simulink library "ammclib_bam_S32K14x"  (R2016a)
settings: Solver=VariableStepAuto  SolverMode=SingleTasking  StartTime=0.0  StopTime=10.0  RelTol=1e-3
undefined symbols (not defined in the file or in its folder): f16A1, f16A2, f16ADCMaxError, f16B0, f16B1, f16B2, f16C1, f16CC1, f16CC1sc, f16CC1sc_D, f16CC1sc_Q, f16CC2, f16CC2sc, f16CC2sc_D, f16CC2sc_Q, f16DerivGain, f16EGain, f16FiltCoef, f16HystOff, f16HystOn, f16IGain, f16IntegGain, f16IntegGainFW, f16IntegGainQ, f16Kd, f16Kq, f16Limit, f16LowerLimit, f16LowerLimit_D, f16LowerLimit_Q, f16LowerLimitFW, f16LowerLimitQ, f16ModIndex, f16OutValOff, f16OutValOn, f16PropGain, f16PropGainFW, f16PropGainQ, f16RampDown, f16RampUp, f16UGain, f16UpperLimit, f16UpperLimit_D, f16UpperLimit_Q, f16UpperLimitFW, f16UpperLimitQ, f16WIGain, f32A1, f32A2, f32ADCMaxError, f32B0, f32B1, f32B2, f32C1, f32CC1, f32CC1sc, f32CC1sc_D, f32CC1sc_Q, f32CC2, f32CC2sc ... (+114)
(part 6 of 22)

== system ammclib_bam_S32K14x/AMCLIB/FLT ==
  AMCLIB_BemfObsrvDQ_FLT : Subsystem  TreatAsAtomicUnit=on  mask(AMCLIB_BemfObsrvDQ_FLT){showStates=Hide (faster execution), resetStatesEnable=Pre-set according to the first set of inputs after reset, fltIGain=0, fltUGain=0, fltWIGain=0, fltEGain=0, fltCC1sc_D=0, fltCC2sc_D=0, fltUpperLimit_D=0, fltLowerLimit_D=0, fltCC1sc_Q=0, fltCC2sc_Q=0, fltUpperLimit_Q=0, fltLowerLimit_Q=0}
      mask prompts: showStates "Show internal states"; resetStatesEnable "Internal state after reset"; fltIGain "fltIGain (RL circuit constant)"; fltUGain "fltUGain (Voltage cross-coupling constant)"; fltWIGain "fltWIGain (Angular velocity cross-coupling constant)"; fltEGain "fltEGain (Back-EMF cross-coupling constant)"; fltCC1sc_D "fltCC1sc_D (CC1 coefficient of the D-axis PI controller)"; fltCC2sc_D "fltCC2sc_D (CC2 coefficient of the D-axis PI controller)"; fltUpperLimit_D "fltUpperLimit_D (Upper Limit of the D-axis PI controller)"; fltLowerLimit_D "fltLowerLimit_D (Lower Limit of the D-axis PI controller)"; fltCC1sc_Q "fltCC1sc_Q (CC1 coefficient of the Q-axis PI controller)"; fltCC2sc_Q "fltCC2sc_Q (CC2 coefficient of the Q-axis PI controller)"; fltUpperLimit_Q "fltUpperLimit_Q (Upper Limit of the Q-axis PI controller)"; fltLowerLimit_Q "fltLowerLimit_Q (Lower Limit of the Q-axis PI controller)"
      mask help: PMSM back-EMF observer DQ in single precision floating-point implementation. This block supports re-initialization of the internal state during simulation. If the block is reset, the observer will align with the motor's position and speed measured in the next time step. This allows seamless on-the-fly transition to the closed-loop control. Refer to the AMMCLIB User's Guide for further details.
      mask init:
      | if ~evalin('base','exist(''tS8'',''var'')')
      |   if (2 ~= exist('SWLIBS_Typedefs.mat','file'))
      |       error('File SWLIBS_Typedefs.mat is not on the Matlab path. Please add the AMMCLIB "bam" folder in the Matlab Search Path.');
      |   else
      |       evalin('base', 'load(''SWLIBS_Typedefs.mat'')');
      |   end
      | end
      | if showStates == 1
      |     % hidden state variables
      |     if strcmp(get_param([gcb '/fltIGain'], 'BlockType'), 'Inport')
      |         posblk = get_param(gcb, 'Position');
      | 
      |         pos = get_param(    [gcb, '/fltIGain'], 'Position');
      |         orient = get_param( [gcb, '/fltIGain'], 'Orientation');
      |         delete_block(       [gcb, '/fltIGain']);
      |         add_block('built-in/Ground', [gcb, '/fltIGain'], 'Position', pos, 'Orientation', orient);
      | 
      |         pos = get_param(    [gcb, '/fltUGain'], 'Position');
      |         orient = get_param( [gcb, '/fltUGain'], 'Orientation');
      |         delete_block(       [gcb, '/fltUGain']);
      |         add_block('built-in/Ground', [gcb, '/fltUGain'], 'Position', pos, 'Orientation', orient);
      | 
      |         pos = get_param(    [gcb, '/fltWIGain'], 'Position');
      |         orient = get_param( [gcb, '/fltWIGain'], 'Orientation');
      |         delete_block(       [gcb, '/fltWIGain']);
      |         add_block('built-in/Ground', [gcb, '/fltWIGain'], 'Position', pos, 'Orientation', orient);
      | 
      |         pos = get_param(    [gcb, '/fltEGain'], 'Position');
      |         orient = get_param( [gcb, '/fltEGain'], 'Orientation');
      |         delete_block(       [gcb, '/fltEGain']);
      |         add_block('built-in/Ground', [gcb, '/fltEGain'], 'Position', pos, 'Orientation', orient);
      | 
      |         pos = get_param(    [gcb, '/fltCC1sc_D'], 'Position');
      |         orient = get_param( [gcb, '/fltCC1sc_D'], 'Orientation');
      |         delete_block(       [gcb, '/fltCC1sc_D']);
      |         add_block('built-in/Ground', [gcb, '/fltCC1sc_D'], 'Position', pos, 'Orientation', orient);
      | 
      |         pos = get_param(    [gcb, '/fltCC2sc_D'], 'Position');
      |         orient = get_param( [gcb, '/fltCC2sc_D'], 'Orientation');
      |         delete_block(       [gcb, '/fltCC2sc_D']);
      |         add_block('built-in/Ground', [gcb, '/fltCC2sc_D'], 'Position', pos, 'Orientation', orient);
      | 
      |         pos = get_param(    [gcb, '/fltUpperLimit_D'], 'Position');
      |         orient = get_param( [gcb, '/fltUpperLimit_D'], 'Orientation');
      |         delete_block(       [gcb, '/fltUpperLimit_D']);
      |         add_block('built-in/Ground', [gcb, '/fltUpperLimit_D'], 'Position', pos, 'Orientation', orient);
      | 
      |         pos = get_param(    [gcb, '/fltLowerLimit_D'], 'Position');
      |         orient = get_param( [gcb, '/fltLowerLimit_D'], 'Orientation');
      |         delete_block(       [gcb, '/fltLowerLimit_D']);
      |         add_block('built-in/Ground', [gcb, '/fltLowerLimit_D'], 'Position', pos, 'Orientation', orient);
      | 
      |         pos = get_param(    [gcb, '/fltCC1sc_Q'], 'Position');
      |         orient = get_param( [gcb, '/fltCC1sc_Q'], 'Orientation');
      |         delete_block(       [gcb, '/fltCC1sc_Q']);
      |         add_block('built-in/Ground', [gcb, '/fltCC1sc_Q'], 'Position', pos, 'Orientation', orient);
      | 
      |         pos = get_param(    [gcb, '/fltCC2sc_Q'], 'Position');
      |         orient = get_param( [gcb, '/fltCC2sc_Q'], 'Orientation');
      |         delete_block(       [gcb, '/fltCC2sc_Q']);
      |         add_block('built-in/Ground', [gcb, '/fltCC2sc_Q'], 'Position', pos, 'Orientation', orient);
      | 
      |         pos = get_param(    [gcb, '/fltUpperLimit_Q'], 'Position');
      |         orient = get_param( [gcb, '/fltUpperLimit_Q'], 'Orientation');
      |         delete_block(       [gcb, '/fltUpperLimit_Q']);
      |         add_block('built-in/Ground', [gcb, '/fltUpperLimit_Q'], 'Position', pos, 'Orientation', orient);
      | 
      |         pos = get_param(    [gcb, '/fltLowerLimit_Q'], 'Position');
      |         orient = get_param( [gcb, '/fltLowerLimit_Q'], 'Orientation');
      |         delete_block(       [gcb, '/fltLowerLimit_Q']);
      |         add_block('built-in/Ground', [gcb, '/fltLowerLimit_Q'], 'Position', pos, 'Orientation', orient);
      | 
      |         pos = get_param(    [gcb, '/fltAcc_D'], 'Position');
      |         orient = get_param( [gcb, '/fltAcc_D'], 'Orientation');
      |         delete_block(       [gcb, '/fltAcc_D']);
      |         add_block('built-in/Ground', [gcb, '/fltAcc_D'], 'Position', pos, 'Orientation', orient);
      | 
      |         pos = get_param(    [gcb, '/fltInErrK1_D'], 'Position');
      |         orient = get_param( [gcb, '/fltInErrK1_D'], 'Orientation');
      |         delete_block(       [gcb, '/fltInErrK1_D']);
      |         add_block('built-in/Ground', [gcb, '/fltInErrK1_D'], 'Position', pos, 'Orientation', orient);
      | 
      |         pos = get_param(    [gcb, '/fltAcc_Q'], 'Position');
      |         orient = get_param( [gcb, '/fltAcc_Q'], 'Orientation');
      |         delete_block(       [gcb, '/fltAcc_Q']);
      |         add_block('built-in/Ground', [gcb, '/fltAcc_Q'], 'Position', pos, 'Orientation', orient);
      | 
      |         pos = get_param(    [gcb, '/fltInErrK1_Q'], 'Position');
      |         orient = get_param( [gcb, '/fltInErrK1_Q'], 'Orientation');
      |         delete_block(       [gcb, '/fltInErrK1_Q']);
      |         add_block('built-in/Ground', [gcb, '/fltInErrK1_Q'], 'Position', pos, 'Orientation', orient);
      | 
      |         pos = get_param(    [gcb, '/fltIObsrvIn_1_D'], 'Position');
      |         orient = get_param( [gcb, '/fltIObsrvIn_1_D'], 'Orientation');
      |         delete_block(       [gcb, '/fltIObsrvIn_1_D']);
      |         add_block('built-in/Ground', [gcb, '/fltIObsrvIn_1_D'], 'Position', pos, 'Orientation', orient);
      | 
      |         pos = get_param(    [gcb, '/fltIObsrvIn_1_Q'], 'Position');
      |         orient = get_param( [gcb, '/fltIObsrvIn_1_Q'], 'Orientation');
      |         delete_block(       [gcb, '/fltIObsrvIn_1_Q']);
      |         add_block('built-in/Ground', [gcb, '/fltIObsrvIn_1_Q'], 'Position', pos, 'Orientation', orient);
      | 
      |         pos = get_param(    [gcb, '/fltIObsrv_D'], 'Position');
      |         orient = get_param( [gcb, '/fltIObsrv_D'], 'Orientation');
      |         delete_block(       [gcb, '/fltIObsrv_D']);
      |         add_block('built-in/Ground', [gcb, '/fltIObsrv_D'], 'Position', pos, 'Orientation', orient);
      | 
      |         pos = get_param(    [gcb, '/fltIObsrv_Q'], 'Position');
      |         orient = get_param( [gcb, '/fltIObsrv_Q'], 'Orientation');
      |         delete_block(       [gcb, '/fltIObsrv_Q']);
      |         add_block('built-in/Ground', [gcb, '/fltIObsrv_Q'], 'Position', pos, 'Orientation', orient);
      | 
      | 
      |         pos = get_param(    [gcb '/fltEObsrv_D_Out'], 'Position');
      |         orient = get_param( [gcb '/fltEObsrv_D_Out'], 'Orientation');
      |         delete_block(       [gcb '/fltEObsrv_D_Out']);
      |         add_block('built-in/Terminator', [gcb '/fltEObsrv_D_Out'], 'Position', pos, 'Orientation', orient);
      | 
      |         pos = get_param(    [gcb '/fltEObsrv_Q_Out'], 'Position');
      |         orient = get_param( [gcb '/fltEObsrv_Q_Out'], 'Orientation');
      |         delete_block(       [gcb '/fltEObsrv_Q_Out']);
      |         add_block('built-in/Terminator', [gcb '/fltEObsrv_Q_Out'], 'Position', pos, 'Orientation', orient);
      | 
      |         pos = get_param(    [gcb '/fltAcc_D_Out'], 'Position');
      |         orient = get_param( [gcb '/fltAcc_D_Out'], 'Orientation');
      |         delete_block(       [gcb '/fltAcc_D_Out']);
      |         add_block('built-in/Terminator', [gcb '/fltAcc_D_Out'], 'Position', pos, 'Orientation', orient);
      | 
      |         pos = get_param(    [gcb '/fltInErrK1_D_Out'], 'Position');
      |         orient = get_param( [gcb '/fltInErrK1_D_Out'], 'Orientation');
      |         delete_block(       [gcb '/fltInErrK1_D_Out']);
      |         add_block('built-in/Terminator', [gcb '/fltInErrK1_D_Out'], 'Position', pos, 'Orientation', orient);
      | 
      |         pos = get_param(    [gcb '/fltAcc_Q_Out'], 'Position');
      |         orient = get_param( [gcb '/fltAcc_Q_Out'], 'Orientation');
      |         delete_block(       [gcb '/fltAcc_Q_Out']);
      |         add_block('built-in/Terminator', [gcb '/fltAcc_Q_Out'], 'Position', pos, 'Orientation', orient);
      | 
      |         pos = get_param(    [gcb '/fltInErrK1_Q_Out'], 'Position');
      |         orient = get_param( [gcb '/fltInErrK1_Q_Out'], 'Orientation');
      |         delete_block(       [gcb '/fltInErrK1_Q_Out']);
      |         add_block('built-in/Terminator', [gcb '/fltInErrK1_Q_Out'], 'Position', pos, 'Orientation', orient);
      | 
      |         pos = get_param(    [gcb '/fltIObsrvIn_1_D_Out'], 'Position');
      |         orient = get_param( [gcb '/fltIObsrvIn_1_D_Out'], 'Orientation');
      |         delete_block(       [gcb '/fltIObsrvIn_1_D_Out']);
      |         add_block('built-in/Terminator', [gcb '/fltIObsrvIn_1_D_Out'], 'Position', pos, 'Orientation', orient);
      | 
      |         pos = get_param(    [gcb '/fltIObsrvIn_1_Q_Out'], 'Position');
      |         orient = get_param( [gcb '/fltIObsrvIn_1_Q_Out'], 'Orientation');
      |         delete_block(       [gcb '/fltIObsrvIn_1_Q_Out']);
      |         add_block('built-in/Terminator', [gcb '/fltIObsrvIn_1_Q_Out'], 'Position', pos, 'Orientation', orient);
      | 
      |         pos = get_param(    [gcb '/fltIObsrv_D_Out'], 'Position');
      |         orient = get_param( [gcb '/fltIObsrv_D_Out'], 'Orientation');
      |         delete_block(       [gcb '/fltIObsrv_D_Out']);
      |         add_block('built-in/Terminator', [gcb '/fltIObsrv_D_Out'], 'Position', pos, 'Orientation', orient);
      | 
      |         pos = get_param(    [gcb '/fltIObsrv_Q_Out'], 'Position');
      |         orient = get_param( [gcb '/fltIObsrv_Q_Out'], 'Orientation');
      |         delete_block(       [gcb '/fltIObsrv_Q_Out']);
      |         add_block('built-in/Terminator', [gcb '/fltIObsrv_Q_Out'], 'Position', pos, 'Orientation', orient);
      | 
      | 
      |         set_param([gcb '/pIAB'], 'Port', '1');
      |         set_param([gcb '/pUAB'], 'Port', '2');
      |         set_param([gcb '/fltVelocity'], 'Port', '3');
      |         set_param([gcb '/fltPhase'], 'Port', '4');
      | 
      |         set_param([gcb '/fltPhaseErr'], 'Port', '1');
      | 
      |         set_param(gcb,'MaskEnables',{'on','on','on','on','on','on','on','on','on','on','on','on','on','on'});
      | 
      |         if (posblk(4) - posblk(2)) > 125
      |           height = 125;
      |           set_param(gcb,'Position',[posblk(1), posblk(2), posblk(3), posblk(2)+height])
      |         end
      |     end
      | else
      |     % shown state variables
      |     if strcmp(get_param([gcb '/fltIGain'], 'BlockType'), 'Ground')
      |         posblk = get_param(gcb, 'Position');
      | 
      |         pos = get_param(    [gcb, '/fltIGain'], 'Position');
      |         orient = get_param( [gcb, '/fltIGain'], 'Orientation');
      |         delete_block(       [gcb, '/fltIGain']);
      |         add_block('built-in/Inport', [gcb, '/fltIGain'], 'Position', pos, 'Orientation', orient, 'OutDataTypeStr', 'single');
      | 
      |         pos = get_param(    [gcb, '/fltUGain'], 'Position');
      |         orient = get_param( [gcb, '/fltUGain'], 'Orientation');
      |         delete_block(       [gcb, '/fltUGain']);
      |         add_block('built-in/Inport', [gcb, '/fltUGain'], 'Position', pos, 'Orientation', orient, 'OutDataTypeStr', 'single');
      | 
      |         pos = get_param(    [gcb, '/fltWIGain'], 'Position');
      |         orient = get_param( [gcb, '/fltWIGain'], 'Orientation');
      |         delete_block(       [gcb, '/fltWIGain']);
      |         add_block('built-in/Inport', [gcb, '/fltWIGain'], 'Position', pos, 'Orientation', orient, 'OutDataTypeStr', 'single');
      | 
      |         pos = get_param(    [gcb, '/fltEGain'], 'Position');
      |         orient = get_param( [gcb, '/fltEGain'], 'Orientation');
      |         delete_block(       [gcb, '/fltEGain']);
      |         add_block('built-in/Inport', [gcb, '/fltEGain'], 'Position', pos, 'Orientation', orient, 'OutDataTypeStr', 'single');
      | 
      |         pos = get_param(    [gcb, '/fltCC1sc_D'], 'Position');
      |         orient = get_param( [gcb, '/fltCC1sc_D'], 'Orientation');
      |         delete_block(       [gcb, '/fltCC1sc_D']);
      |         add_block('built-in/Inport', [gcb, '/fltCC1sc_D'], 'Position', pos, 'Orientation', orient, 'OutDataTypeStr', 'single');
      | 
      |         pos = get_param(    [gcb, '/fltCC2sc_D'], 'Position');
      |         orient = get_param( [gcb, '/fltCC2sc_D'], 'Orientation');
      |         delete_block(       [gcb, '/fltCC2sc_D']);
      |         add_block('built-in/Inport', [gcb, '/fltCC2sc_D'], 'Position', pos, 'Orientation', orient, 'OutDataTypeStr', 'single');
      | 
      |         pos = get_param(    [gcb, '/fltUpperLimit_D'], 'Position');
      |         orient = get_param( [gcb, '/fltUpperLimit_D'], 'Orientation');
      |         delete_block(       [gcb, '/fltUpperLimit_D']);
      |         add_block('built-in/Inport', [gcb, '/fltUpperLimit_D'], 'Position', pos, 'Orientation', orient, 'OutDataTypeStr', 'single');
      | 
      |         pos = get_param(    [gcb, '/fltLowerLimit_D'], 'Position');
      |         orient = get_param( [gcb, '/fltLowerLimit_D'], 'Orientation');
      |         delete_block(       [gcb, '/fltLowerLimit_D']);
      |         add_block('built-in/Inport', [gcb, '/fltLowerLimit_D'], 'Position', pos, 'Orientation', orient, 'OutDataTypeStr', 'single');
      | 
      |         pos = get_param(    [gcb, '/fltCC1sc_Q'], 'Position');
      |         orient = get_param( [gcb, '/fltCC1sc_Q'], 'Orientation');
      |         delete_block(       [gcb, '/fltCC1sc_Q']);
      |         add_block('built-in/Inport', [gcb, '/fltCC1sc_Q'], 'Position', pos, 'Orientation', orient, 'OutDataTypeStr', 'single');
      | 
      |         pos = get_param(    [gcb, '/fltCC2sc_Q'], 'Position');
      |         orient = get_param( [gcb, '/fltCC2sc_Q'], 'Orientation');
      |         delete_block(       [gcb, '/fltCC2sc_Q']);
      |         add_block('built-in/Inport', [gcb, '/fltCC2sc_Q'], 'Position', pos, 'Orientation', orient, 'OutDataTypeStr', 'single');
      | 
      |         pos = get_param(    [gcb, '/fltUpperLimit_Q'], 'Position');
      |         orient = get_param( [gcb, '/fltUpperLimit_Q'], 'Orientation');
      |         delete_block(       [gcb, '/fltUpperLimit_Q']);
      |         add_block('built-in/Inport', [gcb, '/fltUpperLimit_Q'], 'Position', pos, 'Orientation', orient, 'OutDataTypeStr', 'single');
      | 
      |         pos = get_param(    [gcb, '/fltLowerLimit_Q'], 'Position');
      |         orient = get_param( [gcb, '/fltLowerLimit_Q'], 'Orientation');
      |         delete_block(       [gcb, '/fltLowerLimit_Q']);
      |         add_block('built-in/Inport', [gcb, '/fltLowerLimit_Q'], 'Position', pos, 'Orientation', orient, 'OutDataTypeStr', 'single');
      | 
      |         pos = get_param(    [gcb, '/fltAcc_D'], 'Position');
      |         orient = get_param( [gcb, '/fltAcc_D'], 'Orientation');
      |         delete_block(       [gcb, '/fltAcc_D']);
      |         add_block('built-in/Inport', [gcb, '/fltAcc_D'], 'Position', pos, 'Orientation', orient, 'OutDataTypeStr', 'single');
      | 
      |         pos = get_param(    [gcb, '/fltInErrK1_D'], 'Position');
      |         orient = get_param( [gcb, '/fltInErrK1_D'], 'Orientation');
      |         delete_block(       [gcb, '/fltInErrK1_D']);
      |         add_block('built-in/Inport', [gcb, '/fltInErrK1_D'], 'Position', pos, 'Orientation', orient, 'OutDataTypeStr', 'single');
      | 
      |         pos = get_param(    [gcb, '/fltAcc_Q'], 'Position');
      |         orient = get_param( [gcb, '/fltAcc_Q'], 'Orientation');
      |         delete_block(       [gcb, '/fltAcc_Q']);
      |         add_block('built-in/Inport', [gcb, '/fltAcc_Q'], 'Position', pos, 'Orientation', orient, 'OutDataTypeStr', 'single');
      | 
      |         pos = get_param(    [gcb, '/fltInErrK1_Q'], 'Position');
      |         orient = get_param( [gcb, '/fltInErrK1_Q'], 'Orientation');
      |         delete_block(       [gcb, '/fltInErrK1_Q']);
      |         add_block('built-in/Inport', [gcb, '/fltInErrK1_Q'], 'Position', pos, 'Orientation', orient, 'OutDataTypeStr', 'single');
      | 
      |         pos = get_param(    [gcb, '/fltIObsrvIn_1_D'], 'Position');
      |         orient = get_param( [gcb, '/fltIObsrvIn_1_D'], 'Orientation');
      |         delete_block(       [gcb, '/fltIObsrvIn_1_D']);
      |         add_block('built-in/Inport', [gcb, '/fltIObsrvIn_1_D'], 'Position', pos, 'Orientation', orient, 'OutDataTypeStr', 'single');
      | 
      |         pos = get_param(    [gcb, '/fltIObsrvIn_1_Q'], 'Position');
      |         orient = get_param( [gcb, '/fltIObsrvIn_1_Q'], 'Orientation');
      |         delete_block(       [gcb, '/fltIObsrvIn_1_Q']);
      |         add_block('built-in/Inport', [gcb, '/fltIObsrvIn_1_Q'], 'Position', pos, 'Orientation', orient, 'OutDataTypeStr', 'single');
      | 
      |         pos = get_param(    [gcb, '/fltIObsrv_D'], 'Position');
      |         orient = get_param( [gcb, '/fltIObsrv_D'], 'Orientation');
      |         delete_block(       [gcb, '/fltIObsrv_D']);
      |         add_block('built-in/Inport', [gcb, '/fltIObsrv_D'], 'Position', pos, 'Orientation', orient, 'OutDataTypeStr', 'single');
      | 
      |         pos = get_param(    [gcb, '/fltIObsrv_Q'], 'Position');
      |         orient = get_param( [gcb, '/fltIObsrv_Q'], 'Orientation');
      |         delete_block(       [gcb, '/fltIObsrv_Q']);
      |         add_block('built-in/Inport', [gcb, '/fltIObsrv_Q'], 'Position', pos, 'Orientation', orient, 'OutDataTypeStr', 'single');
      | 
      | 
      |         pos = get_param(    [gcb '/fltEObsrv_D_Out'], 'Position');
      |         orient = get_param( [gcb '/fltEObsrv_D_Out'], 'Orientation');
      |         delete_block(       [gcb '/fltEObsrv_D_Out']);
      |         add_block('built-in/Outport', [gcb '/fltEObsrv_D_Out'], 'Position', pos, 'Orientation', orient);
      | 
      |         pos = get_param(    [gcb '/fltEObsrv_Q_Out'], 'Position');
      |         orient = get_param( [gcb '/fltEObsrv_Q_Out'], 'Orientation');
      |         delete_block(       [gcb '/fltEObsrv_Q_Out']);
      |         add_block('built-in/Outport', [gcb '/fltEObsrv_Q_Out'], 'Position', pos, 'Orientation', orient);
      | 
      |         pos = get_param(    [gcb '/fltAcc_D_Out'], 'Position');
      |         orient = get_param( [gcb '/fltAcc_D_Out'], 'Orientation');
      |         delete_block(       [gcb '/fltAcc_D_Out']);
      |         add_block('built-in/Outport', [gcb '/fltAcc_D_Out'], 'Position', pos, 'Orientation', orient);
      | 
      |         pos = get_param(    [gcb '/fltInErrK1_D_Out'], 'Position');
      |         orient = get_param( [gcb '/fltInErrK1_D_Out'], 'Orientation');
      |         delete_block(       [gcb '/fltInErrK1_D_Out']);
      |         add_block('built-in/Outport', [gcb '/fltInErrK1_D_Out'], 'Position', pos, 'Orientation', orient);
      | 
      |         pos = get_param(    [gcb '/fltAcc_Q_Out'], 'Position');
      |         orient = get_param( [gcb '/fltAcc_Q_Out'], 'Orientation');
      |         delete_block(       [gcb '/fltAcc_Q_Out']);
      |         add_block('built-in/Outport', [gcb '/fltAcc_Q_Out'], 'Position', pos, 'Orientation', orient);
      | 
      |         pos = get_param(    [gcb '/fltInErrK1_Q_Out'], 'Position');
      |         orient = get_param( [gcb '/fltInErrK1_Q_Out'], 'Orientation');
      |         delete_block(       [gcb '/fltInErrK1_Q_Out']);
      |         add_block('built-in/Outport', [gcb '/fltInErrK1_Q_Out'], 'Position', pos, 'Orientation', orient);
      | 
      |         pos = get_param(    [gcb '/fltIObsrvIn_1_D_Out'], 'Position');
      |         orient = get_param( [gcb '/fltIObsrvIn_1_D_Out'], 'Orientation');
      |         delete_block(       [gcb '/fltIObsrvIn_1_D_Out']);
      |         add_block('built-in/Outport', [gcb '/fltIObsrvIn_1_D_Out'], 'Position', pos, 'Orientation', orient);
      | 
      |         pos = get_param(    [gcb '/fltIObsrvIn_1_Q_Out'], 'Position');
      |         orient = get_param( [gcb '/fltIObsrvIn_1_Q_Out'], 'Orientation');
      |         delete_block(       [gcb '/fltIObsrvIn_1_Q_Out']);
      |         add_block('built-in/Outport', [gcb '/fltIObsrvIn_1_Q_Out'], 'Position', pos, 'Orientation', orient);
      | 
      |         pos = get_param(    [gcb '/fltIObsrv_D_Out'], 'Position');
      |         orient = get_param( [gcb '/fltIObsrv_D_Out'], 'Orientation');
      |         delete_block(       [gcb '/fltIObsrv_D_Out']);
      |         add_block('built-in/Outport', [gcb '/fltIObsrv_D_Out'], 'Position', pos, 'Orientation', orient);
      | 
      |         pos = get_param(    [gcb '/fltIObsrv_Q_Out'], 'Position');
      |         orient = get_param( [gcb '/fltIObsrv_Q_Out'], 'Orientation');
      |         delete_block(       [gcb '/fltIObsrv_Q_Out']);
      |         add_block('built-in/Outport', [gcb '/fltIObsrv_Q_Out'], 'Position', pos, 'Orientation', orient);
      | 
      | 
      |         set_param([gcb '/pIAB'], 'Port', '1');
      |         set_param([gcb '/pUAB'], 'Port', '2');
      |         set_param([gcb '/fltVelocity'], 'Port', '3');
      |         set_param([gcb '/fltPhase'], 'Port', '4');
      |         set_param([gcb '/fltIGain'], 'Port', '5');
      |         set_param([gcb '/fltUGain'], 'Port', '6');
      |         set_param([gcb '/fltWIGain'], 'Port', '7');
      |         set_param([gcb '/fltEGain'], 'Port', '8');
      |         set_param([gcb '/fltCC1sc_D'], 'Port', '9');
      |         set_param([gcb '/fltCC2sc_D'], 'Port', '10');
      |         set_param([gcb '/fltUpperLimit_D'], 'Port', '11');
      |         set_param([gcb '/fltLowerLimit_D'], 'Port', '12');
      |         set_param([gcb '/fltCC1sc_Q'], 'Port', '13');
      |         set_param([gcb '/fltCC2sc_Q'], 'Port', '14');
      |         set_param([gcb '/fltUpperLimit_Q'], 'Port', '15');
      |         set_param([gcb '/fltLowerLimit_Q'], 'Port', '16');
      |         set_param([gcb '/fltAcc_D'], 'Port', '17');
      |         set_param([gcb '/fltInErrK1_D'], 'Port', '18');
      |         set_param([gcb '/fltAcc_Q'], 'Port', '19');
      |         set_param([gcb '/fltInErrK1_Q'], 'Port', '20');
      |         set_param([gcb '/fltIObsrvIn_1_D'], 'Port', '21');
      |         set_param([gcb '/fltIObsrvIn_1_Q'], 'Port', '22');
      |         set_param([gcb '/fltIObsrv_D'], 'Port', '23');
      |         set_param([gcb '/fltIObsrv_Q'], 'Port', '24');
      | 
      |         set_param([gcb '/fltPhaseErr'], 'Port', '1');
      |         set_param([gcb '/fltEObsrv_D_Out'], 'Port', '2');
      |         set_param([gcb '/fltEObsrv_Q_Out'], 'Port', '3');
      |         set_param([gcb '/fltAcc_D_Out'], 'Port', '4');
      |         set_param([gcb '/fltInErrK1_D_Out'], 'Port', '5');
      |         set_param([gcb '/fltAcc_Q_Out'], 'Port', '6');
      |         set_param([gcb '/fltInErrK1_Q_Out'], 'Port', '7');
      |         set_param([gcb '/fltIObsrvIn_1_D_Out'], 'Port', '8');
      |         set_param([gcb '/fltIObsrvIn_1_Q_Out'], 'Port', '9');
      |         set_param([gcb '/fltIObsrv_D_Out'], 'Port', '10');
      |         set_param([gcb '/fltIObsrv_Q_Out'], 'Port', '11');
      | 
      |         set_param(gcb,'MaskEnables',{'on','on','off','off','off','off','off','off','off','off','off','off','off','off'});
      | 
      |         if (posblk(4) - posblk(2)) < 625
      |           height = 625;
      |           set_param(gcb,'Position',[posblk(1), posblk(2), posblk(3), posblk(2)+height])
      |         end
      |     end
      | end
      settings: RTWSystemCode=Inline
      mask Help: web([fileparts(which('ammclib_bam_S32K14x.slx')) '/../doc/S32K14XMCLUG.pdf'], '-browser')
      mask TypeOptions showStates: Hide (faster execution) | Show (allows debugging; connect feedback loops manually)
      mask Callback showStates:
      | maskStr = get_param(gcb,'showStates');
      | if strcmp(maskStr,'Hide (faster execution)'),
      |     set_param(gcb,'MaskEnables',{'on','on','on','on','on','on','on','on','on','on','on','on','on','on'});
      | else
      |     set_param(gcb,'MaskEnables',{'on','on','off','off','off','off','off','off','off','off','off','off','off','off'});
      | end
      mask TypeOptions resetStatesEnable: Pre-set according to the first set of inputs after reset | Clear to zero
      mask Display:
      | color('black');
      | pos = get_param(gcb, 'Position');
      | width = pos(3) - pos(1);
      | height = pos(4) - pos(2);
      | tX=width/2;
      | tY=height - 25;
      | color('black');
      | text(tX,tY, 'AMCLIB_BemfObsrvDQ_FLT', 'horizontalAlignment', 'center');
      | if showStates == 2
      |   color('red');
      |   text(tX,tY - 20, ['debugging mode' char(13) char(10) '(limited performance)'], 'horizontalAlignment', 'center');
      | end
  AMCLIB_CurrentLoop_FLT : Subsystem  TreatAsAtomicUnit=on  mask(AMCLIB_CurrentLoop_FLT){showStates=Hide (faster execution), resetStatesEnable=Pre-set according to the first set of inputs after reset, fltCC1sc_D=0, fltCC2sc_D=0, fltCC1sc_Q=0, fltCC2sc_Q=0}
      mask prompts: showStates "Show internal states"; resetStatesEnable "Internal state after reset"; fltCC1sc_D "fltCC1sc_D (CC1 coefficient of the D-axis PI controller)"; fltCC2sc_D "fltCC2sc_D (CC2 coefficient of the D-axis PI controller)"; fltCC1sc_Q "fltCC1sc_Q (CC1 coefficient of the Q-axis PI controller)"; fltCC2sc_Q "fltCC2sc_Q (CC2 coefficient of the Q-axis PI controller)"
      mask help: Current control loop of the PMSM field-oriented control algorithm in single precision floating-point implementation. This block supports re-initialization of the internal state during simulation. If the block is reset, the outputs of the PI controllers will be aligned with the inputs fltControllerPIrAWDOut_preset and fltControllerPIrAWQOut_preset. Refer to the AMMCLIB User's Guide for further details.
      mask init:
      | if ~evalin('base','exist(''tS8'',''var'')')
      |   if (2 ~= exist('SWLIBS_Typedefs.mat','file'))
      |       error('File SWLIBS_Typedefs.mat is not on the Matlab path. Please add the AMMCLIB "bam" folder in the Matlab Search Path.');
      |   else
      |       evalin('base', 'load(''SWLIBS_Typedefs.mat'')');
      |   end
      | end
      | if showStates == 1
      |     % hidden state variables
      |     if strcmp(get_param([gcb '/fltCC1sc_D'], 'BlockType'), 'Inport')
      |         posblk = get_param(gcb, 'Position');
      | 
      |         pos = get_param(    [gcb, '/fltCC1sc_D'], 'Position');
      |         orient = get_param( [gcb, '/fltCC1sc_D'], 'Orientation');
      |         delete_block(       [gcb, '/fltCC1sc_D']);
      |         add_block('built-in/Ground', [gcb, '/fltCC1sc_D'], 'Position', pos, 'Orientation', orient);
      | 
      |         pos = get_param(    [gcb, '/fltCC2sc_D'], 'Position');
      |         orient = get_param( [gcb, '/fltCC2sc_D'], 'Orientation');
      |         delete_block(       [gcb, '/fltCC2sc_D']);
      |         add_block('built-in/Ground', [gcb, '/fltCC2sc_D'], 'Position', pos, 'Orientation', orient);
      | 
      |         pos = get_param(    [gcb, '/fltCC1sc_Q'], 'Position');
      |         orient = get_param( [gcb, '/fltCC1sc_Q'], 'Orientation');
      |         delete_block(       [gcb, '/fltCC1sc_Q']);
      |         add_block('built-in/Ground', [gcb, '/fltCC1sc_Q'], 'Position', pos, 'Orientation', orient);
      | 
      |         pos = get_param(    [gcb, '/fltCC2sc_Q'], 'Position');
      |         orient = get_param( [gcb, '/fltCC2sc_Q'], 'Orientation');
      |         delete_block(       [gcb, '/fltCC2sc_Q']);
      |         add_block('built-in/Ground', [gcb, '/fltCC2sc_Q'], 'Position', pos, 'Orientation', orient);
      | 
      |         pos = get_param(    [gcb, '/fltAcc_D'], 'Position');
      |         orient = get_param( [gcb, '/fltAcc_D'], 'Orientation');
      |         delete_block(       [gcb, '/fltAcc_D']);
      |         add_block('built-in/Ground', [gcb, '/fltAcc_D'], 'Position', pos, 'Orientation', orient);
      | 
      |         pos = get_param(    [gcb, '/fltInErrK1_D'], 'Position');
      |         orient = get_param( [gcb, '/fltInErrK1_D'], 'Orientation');
      |         delete_block(       [gcb, '/fltInErrK1_D']);
      |         add_block('built-in/Ground', [gcb, '/fltInErrK1_D'], 'Position', pos, 'Orientation', orient);
      | 
      |         pos = get_param(    [gcb, '/fltAcc_Q'], 'Position');
      |         orient = get_param( [gcb, '/fltAcc_Q'], 'Orientation');
      |         delete_block(       [gcb, '/fltAcc_Q']);
      |         add_block('built-in/Ground', [gcb, '/fltAcc_Q'], 'Position', pos, 'Orientation', orient);
      | 
      |         pos = get_param(    [gcb, '/fltInErrK1_Q'], 'Position');
      |         orient = get_param( [gcb, '/fltInErrK1_Q'], 'Orientation');
      |         delete_block(       [gcb, '/fltInErrK1_Q']);
      |         add_block('built-in/Ground', [gcb, '/fltInErrK1_Q'], 'Position', pos, 'Orientation', orient);
      | 
      | 
      |         pos = get_param(    [gcb '/fltAcc_D_Out'], 'Position');
      |         orient = get_param( [gcb '/fltAcc_D_Out'], 'Orientation');
      |         delete_block(       [gcb '/fltAcc_D_Out']);
      |         add_block('built-in/Terminator', [gcb '/fltAcc_D_Out'], 'Position', pos, 'Orientation', orient);
      | 
      |         pos = get_param(    [gcb '/fltInErrK1_D_Out'], 'Position');
      |         orient = get_param( [gcb '/fltInErrK1_D_Out'], 'Orientation');
      |         delete_block(       [gcb '/fltInErrK1_D_Out']);
      |         add_block('built-in/Terminator', [gcb '/fltInErrK1_D_Out'], 'Position', pos, 'Orientation', orient);
      | 
      |         pos = get_param(    [gcb '/fltAcc_Q_Out'], 'Position');
      |         orient = get_param( [gcb '/fltAcc_Q_Out'], 'Orientation');
      |         delete_block(       [gcb '/fltAcc_Q_Out']);
      |         add_block('built-in/Terminator', [gcb '/fltAcc_Q_Out'], 'Position', pos, 'Orientation', orient);
      | 
      |         pos = get_param(    [gcb '/fltInErrK1_Q_Out'], 'Position');
      |         orient = get_param( [gcb '/fltInErrK1_Q_Out'], 'Orientation');
      |         delete_block(       [gcb '/fltInErrK1_Q_Out']);
      |         add_block('built-in/Terminator', [gcb '/fltInErrK1_Q_Out'], 'Position', pos, 'Orientation', orient);
      | 
      | 
      |         set_param([gcb '/fltUDcBus'], 'Port', '1');
      |         set_param([gcb '/pIDQReq'], 'Port', '2');
      |         set_param([gcb '/pIDQFbck'], 'Port', '3');
      |         set_param([gcb '/fltControllerPIrAWDOut_preset'], 'Port', '4');
      |         set_param([gcb '/fltControllerPIrAWQOut_preset'], 'Port', '5');
      | 
      |         set_param([gcb '/pUDQReq'], 'Port', '1');
      | 
      |         set_param(gcb,'MaskEnables',{'on','on','on','on','on','on'});
      | 
      |         if (posblk(4) - posblk(2)) > 150
      |           height = 150;
      |           set_param(gcb,'Position',[posblk(1), posblk(2), posblk(3), posblk(2)+height])
      |         end
      |     end
      | else
      |     % shown state variables
      |     if strcmp(get_param([gcb '/fltCC1sc_D'], 'BlockType'), 'Ground')
      |         posblk = get_param(gcb, 'Position');
      | 
      |         pos = get_param(    [gcb, '/fltCC1sc_D'], 'Position');
      |         orient = get_param( [gcb, '/fltCC1sc_D'], 'Orientation');
      |         delete_block(       [gcb, '/fltCC1sc_D']);
      |         add_block('built-in/Inport', [gcb, '/fltCC1sc_D'], 'Position', pos, 'Orientation', orient, 'OutDataTypeStr', 'single');
      | 
      |         pos = get_param(    [gcb, '/fltCC2sc_D'], 'Position');
      |         orient = get_param( [gcb, '/fltCC2sc_D'], 'Orientation');
      |         delete_block(       [gcb, '/fltCC2sc_D']);
      |         add_block('built-in/Inport', [gcb, '/fltCC2sc_D'], 'Position', pos, 'Orientation', orient, 'OutDataTypeStr', 'single');
      | 
      |         pos = get_param(    [gcb, '/fltCC1sc_Q'], 'Position');
      |         orient = get_param( [gcb, '/fltCC1sc_Q'], 'Orientation');
      |         delete_block(       [gcb, '/fltCC1sc_Q']);
      |         add_block('built-in/Inport', [gcb, '/fltCC1sc_Q'], 'Position', pos, 'Orientation', orient, 'OutDataTypeStr', 'single');
      | 
      |         pos = get_param(    [gcb, '/fltCC2sc_Q'], 'Position');
      |         orient = get_param( [gcb, '/fltCC2sc_Q'], 'Orientation');
      |         delete_block(       [gcb, '/fltCC2sc_Q']);
      |         add_block('built-in/Inport', [gcb, '/fltCC2sc_Q'], 'Position', pos, 'Orientation', orient, 'OutDataTypeStr', 'single');
      | 
      |         pos = get_param(    [gcb, '/fltAcc_D'], 'Position');
      |         orient = get_param( [gcb, '/fltAcc_D'], 'Orientation');
      |         delete_block(       [gcb, '/fltAcc_D']);
      |         add_block('built-in/Inport', [gcb, '/fltAcc_D'], 'Position', pos, 'Orientation', orient, 'OutDataTypeStr', 'single');
      | 
      |         pos = get_param(    [gcb, '/fltInErrK1_D'], 'Position');
      |         orient = get_param( [gcb, '/fltInErrK1_D'], 'Orientation');
      |         delete_block(       [gcb, '/fltInErrK1_D']);
      |         add_block('built-in/Inport', [gcb, '/fltInErrK1_D'], 'Position', pos, 'Orientation', orient, 'OutDataTypeStr', 'single');
      | 
      |         pos = get_param(    [gcb, '/fltAcc_Q'], 'Position');
      |         orient = get_param( [gcb, '/fltAcc_Q'], 'Orientation');
      |         delete_block(       [gcb, '/fltAcc_Q']);
      |         add_block('built-in/Inport', [gcb, '/fltAcc_Q'], 'Position', pos, 'Orientation', orient, 'OutDataTypeStr', 'single');
      | 
      |         pos = get_param(    [gcb, '/fltInErrK1_Q'], 'Position');
      |         orient = get_param( [gcb, '/fltInErrK1_Q'], 'Orientation');
      |         delete_block(       [gcb, '/fltInErrK1_Q']);
      |         add_block('built-in/Inport', [gcb, '/fltInErrK1_Q'], 'Position', pos, 'Orientation', orient, 'OutDataTypeStr', 'single');
      | 
      | 
      |         pos = get_param(    [gcb '/fltAcc_D_Out'], 'Position');
      |         orient = get_param( [gcb '/fltAcc_D_Out'], 'Orientation');
      |         delete_block(       [gcb '/fltAcc_D_Out']);
      |         add_block('built-in/Outport', [gcb '/fltAcc_D_Out'], 'Position', pos, 'Orientation', orient);
      | 
      |         pos = get_param(    [gcb '/fltInErrK1_D_Out'], 'Position');
      |         orient = get_param( [gcb '/fltInErrK1_D_Out'], 'Orientation');
      |         delete_block(       [gcb '/fltInErrK1_D_Out']);
      |         add_block('built-in/Outport', [gcb '/fltInErrK1_D_Out'], 'Position', pos, 'Orientation', orient);
      | 
      |         pos = get_param(    [gcb '/fltAcc_Q_Out'], 'Position');
      |         orient = get_param( [gcb '/fltAcc_Q_Out'], 'Orientation');
      |         delete_block(       [gcb '/fltAcc_Q_Out']);
      |         add_block('built-in/Outport', [gcb '/fltAcc_Q_Out'], 'Position', pos, 'Orientation', orient);
      | 
      |         pos = get_param(    [gcb '/fltInErrK1_Q_Out'], 'Position');
      |         orient = get_param( [gcb '/fltInErrK1_Q_Out'], 'Orientation');
      |         delete_block(       [gcb '/fltInErrK1_Q_Out']);
      |         add_block('built-in/Outport', [gcb '/fltInErrK1_Q_Out'], 'Position', pos, 'Orientation', orient);
      | 
      | 
      |         set_param([gcb '/fltUDcBus'], 'Port', '1');
      |         set_param([gcb '/pIDQReq'], 'Port', '2');
      |         set_param([gcb '/pIDQFbck'], 'Port', '3');
      |         set_param([gcb '/fltControllerPIrAWDOut_preset'], 'Port', '4');
      |         set_param([gcb '/fltControllerPIrAWQOut_preset'], 'Port', '5');
      |         set_param([gcb '/fltCC1sc_D'], 'Port', '6');
      |         set_param([gcb '/fltCC2sc_D'], 'Port', '7');
      |         set_param([gcb '/fltCC1sc_Q'], 'Port', '8');
      |         set_param([gcb '/fltCC2sc_Q'], 'Port', '9');
      |         set_param([gcb '/fltAcc_D'], 'Port', '10');
      |         set_param([gcb '/fltInErrK1_D'], 'Port', '11');
      |         set_param([gcb '/fltAcc_Q'], 'Port', '12');
      |         set_param([gcb '/fltInErrK1_Q'], 'Port', '13');
      | 
      |         set_param([gcb '/pUDQReq'], 'Port', '1');
      |         set_param([gcb '/fltAcc_D_Out'], 'Port', '2');
      |         set_param([gcb '/fltInErrK1_D_Out'], 'Port', '3');
      |         set_param([gcb '/fltAcc_Q_Out'], 'Port', '4');
      |         set_param([gcb '/fltInErrK1_Q_Out'], 'Port', '5');
      | 
      |         set_param(gcb,'MaskEnables',{'on','on','off','off','off','off'});
      | 
      |         if (posblk(4) - posblk(2)) < 350
      |           height = 350;
      |           set_param(gcb,'Position',[posblk(1), posblk(2), posblk(3), posblk(2)+height])
      |         end
      |     end
      | end
      settings: RTWSystemCode=Inline
      mask Help: web([fileparts(which('ammclib_bam_S32K14x.slx')) '/../doc/S32K14XMCLUG.pdf'], '-browser')
      mask TypeOptions showStates: Hide (faster execution) | Show (allows debugging; connect feedback loops manually)
      mask Callback showStates:
      | maskStr = get_param(gcb,'showStates');
      | if strcmp(maskStr,'Hide (faster execution)'),
      |     set_param(gcb,'MaskEnables',{'on','on','on','on','on','on'});
      | else
      |     set_param(gcb,'MaskEnables',{'on','on','off','off','off','off'});
      | end
      mask TypeOptions resetStatesEnable: Pre-set according to the first set of inputs after reset | Clear to zero
      mask Display:
      | color('black');
      | pos = get_param(gcb, 'Position');
      | width = pos(3) - pos(1);
      | height = pos(4) - pos(2);
      | tX=width/2;
      | tY=height - 25;
      | color('black');
      | text(tX,tY, 'AMCLIB_CurrentLoop_FLT', 'horizontalAlignment', 'center');
      | if showStates == 2
      |   color('red');
      |   text(tX,tY - 20, ['debugging mode' char(13) char(10) '(limited performance)'], 'horizontalAlignment', 'center');
      | end
  AMCLIB_FWSpeedLoop_FLT : Subsystem  TreatAsAtomicUnit=on  mask(AMCLIB_FWSpeedLoop_FLT){showStates=Hide (faster execution), resetStatesEnable=Pre-set according to the first set of inputs after reset, showDebugOutputs=Hide, fltUmaxDivImax=0, fltLambdaW=0, fltLambdaFW=0, fltPropGainQ=0, fltIntegGainQ=0, fltLowerLimitQ=0, fltUpperLimitQ=0, fltPropGainFW=0, fltIntegGainFW=0, fltLowerLimitFW=0, fltUpperLimitFW=0, fltRampUp=0, fltRampDown=0}
      mask prompts: showStates "Show internal states"; resetStatesEnable "Internal state after reset"; showDebugOutputs "Show debugging outputs"; fltUmaxDivImax "fltUmaxDivImax (Maximal coil voltage divided by the maximal coil current)"; fltLambdaW "fltLambdaW (velocity GDFLIB_FilterMA - smoothing factor)"; fltLambdaFW "fltLambdaFW (FW GDFLIB_FilterMA - smoothing factor)"; fltPropGainQ "fltPropGainQ (q-axis GFLIB_ControllerPIpAW - proportional gain)"; fltIntegGainQ "fltIntegGainQ (q-axis GFLIB_ControllerPIpAW - integral gain)"; fltLowerLimitQ "fltLowerLimitQ (q-axis GFLIB_ControllerPIpAW - lower limit)"; fltUpperLimitQ "fltUpperLimitQ (q-axis GFLIB_ControllerPIpAW - upper limit)"; fltPropGainFW "fltPropGainFW (FW GFLIB_ControllerPIpAW - proportional gain)"; fltIntegGainFW "fltIntegGainFW (FW GFLIB_ControllerPIpAW - integral gain)"; fltLowerLimitFW "fltLowerLimitFW (FW GFLIB_ControllerPIpAW - lower limit)"; fltUpperLimitFW "fltUpperLimitFW (FW GFLIB_ControllerPIpAW - upper limit)"; fltRampUp "fltRampUp (Ramp up increment coefficient)"; fltRampDown "fltRampDown (Ramp up decrement coefficient)"
      mask help: Speed loop controller with Field Weakening capability for the PMSM field-oriented control algorithm in single precision floating-point implementation. This block supports re-initialization of the internal state during simulation. If the block is reset, the outputs of the MA filters, PI controllers, and the ramp will be aligned with the inputs fltFilterMAWOut_preset, fltFilterMAFWOut_preset, fltControllerPIpAWQOut_preset, fltControllerPIpAWFWOut_preset, and fltRampOut_preset. Refer to the AMMCLIB User's Guide for further details.
      mask init:
      | if ~evalin('base','exist(''tS8'',''var'')')
      |   if (2 ~= exist('SWLIBS_Typedefs.mat','file'))
      |       error('File SWLIBS_Typedefs.mat is not on the Matlab path. Please add the AMMCLIB "bam" folder in the Matlab Search Path.');
      |   else
      |       evalin('base', 'load(''SWLIBS_Typedefs.mat'')');
      |   end
      | end
      | if showStates == 1
      |     % hidden state variables
      |     if strcmp(get_param([gcb '/fltUmaxDivImax'], 'BlockType'), 'Inport')
      |         posblk = get_param(gcb, 'Position');
      | 
      |         pos = get_param(    [gcb, '/fltUmaxDivImax'], 'Position');
      |         orient = get_param( [gcb, '/fltUmaxDivImax'], 'Orientation');
      |         delete_block(       [gcb, '/fltUmaxDivImax']);
      |         add_block('built-in/Ground', [gcb, '/fltUmaxDivImax'], 'Position', pos, 'Orientation', orient);
      | 
      |         pos = get_param(    [gcb, '/fltLambdaW'], 'Position');
      |         orient = get_param( [gcb, '/fltLambdaW'], 'Orientation');
      |         delete_block(       [gcb, '/fltLambdaW']);
      |         add_block('built-in/Ground', [gcb, '/fltLambdaW'], 'Position', pos, 'Orientation', orient);
      | 
      |         pos = get_param(    [gcb, '/fltLambdaFW'], 'Position');
      |         orient = get_param( [gcb, '/fltLambdaFW'], 'Orientation');
      |         delete_block(       [gcb, '/fltLambdaFW']);
      |         add_block('built-in/Ground', [gcb, '/fltLambdaFW'], 'Position', pos, 'Orientation', orient);
      | 
      |         pos = get_param(    [gcb, '/fltPropGainQ'], 'Position');
      |         orient = get_param( [gcb, '/fltPropGainQ'], 'Orientation');
      |         delete_block(       [gcb, '/fltPropGainQ']);
      |         add_block('built-in/Ground', [gcb, '/fltPropGainQ'], 'Position', pos, 'Orientation', orient);
      | 
      |         pos = get_param(    [gcb, '/fltIntegGainQ'], 'Position');
      |         orient = get_param( [gcb, '/fltIntegGainQ'], 'Orientation');
      |         delete_block(       [gcb, '/fltIntegGainQ']);
      |         add_block('built-in/Ground', [gcb, '/fltIntegGainQ'], 'Position', pos, 'Orientation', orient);
      | 
      |         pos = get_param(    [gcb, '/fltLowerLimitQ'], 'Position');
      |         orient = get_param( [gcb, '/fltLowerLimitQ'], 'Orientation');
      |         delete_block(       [gcb, '/fltLowerLimitQ']);
      |         add_block('built-in/Ground', [gcb, '/fltLowerLimitQ'], 'Position', pos, 'Orientation', orient);
      | 
      |         pos = get_param(    [gcb, '/fltUpperLimitQ'], 'Position');
      |         orient = get_param( [gcb, '/fltUpperLimitQ'], 'Orientation');
      |         delete_block(       [gcb, '/fltUpperLimitQ']);
      |         add_block('built-in/Ground', [gcb, '/fltUpperLimitQ'], 'Position', pos, 'Orientation', orient);
      | 
      |         pos = get_param(    [gcb, '/fltPropGainFW'], 'Position');
      |         orient = get_param( [gcb, '/fltPropGainFW'], 'Orientation');
      |         delete_block(       [gcb, '/fltPropGainFW']);
      |         add_block('built-in/Ground', [gcb, '/fltPropGainFW'], 'Position', pos, 'Orientation', orient);
      | 
      |         pos = get_param(    [gcb, '/fltIntegGainFW'], 'Position');
      |         orient = get_param( [gcb, '/fltIntegGainFW'], 'Orientation');
      |         delete_block(       [gcb, '/fltIntegGainFW']);
      |         add_block('built-in/Ground', [gcb, '/fltIntegGainFW'], 'Position', pos, 'Orientation', orient);
      | 
      |         pos = get_param(    [gcb, '/fltLowerLimitFW'], 'Position');
      |         orient = get_param( [gcb, '/fltLowerLimitFW'], 'Orientation');
      |         delete_block(       [gcb, '/fltLowerLimitFW']);
      |         add_block('built-in/Ground', [gcb, '/fltLowerLimitFW'], 'Position', pos, 'Orientation', orient);
      | 
      |         pos = get_param(    [gcb, '/fltUpperLimitFW'], 'Position');
      |         orient = get_param( [gcb, '/fltUpperLimitFW'], 'Orientation');
      |         delete_block(       [gcb, '/fltUpperLimitFW']);
      |         add_block('built-in/Ground', [gcb, '/fltUpperLimitFW'], 'Position', pos, 'Orientation', orient);
      | 
      |         pos = get_param(    [gcb, '/fltRampUp'], 'Position');
      |         orient = get_param( [gcb, '/fltRampUp'], 'Orientation');
      |         delete_block(       [gcb, '/fltRampUp']);
      |         add_block('built-in/Ground', [gcb, '/fltRampUp'], 'Position', pos, 'Orientation', orient);
      | 
      |         pos = get_param(    [gcb, '/fltRampDown'], 'Position');
      |         orient = get_param( [gcb, '/fltRampDown'], 'Orientation');
      |         delete_block(       [gcb, '/fltRampDown']);
      |         add_block('built-in/Ground', [gcb, '/fltRampDown'], 'Position', pos, 'Orientation', orient);
      | 
      |         pos = get_param(    [gcb, '/fltIQReqK_1'], 'Position');
      |         orient = get_param( [gcb, '/fltIQReqK_1'], 'Orientation');
      |         delete_block(       [gcb, '/fltIQReqK_1']);
      |         add_block('built-in/Ground', [gcb, '/fltIQReqK_1'], 'Position', pos, 'Orientation', orient);
      | 
      |         pos = get_param(    [gcb, '/fltAccW'], 'Position');
      |         orient = get_param( [gcb, '/fltAccW'], 'Orientation');
      |         delete_block(       [gcb, '/fltAccW']);
      |         add_block('built-in/Ground', [gcb, '/fltAccW'], 'Position', pos, 'Orientation', orient);
      | 
      |         pos = get_param(    [gcb, '/fltAccFW'], 'Position');
      |         orient = get_param( [gcb, '/fltAccFW'], 'Orientation');
      |         delete_block(       [gcb, '/fltAccFW']);
      |         add_block('built-in/Ground', [gcb, '/fltAccFW'], 'Position', pos, 'Orientation', orient);
      | 
      |         pos = get_param(    [gcb, '/fltIntegPartK_1Q'], 'Position');
      |         orient = get_param( [gcb, '/fltIntegPartK_1Q'], 'Orientation');
      |         delete_block(       [gcb, '/fltIntegPartK_1Q']);
      |         add_block('built-in/Ground', [gcb, '/fltIntegPartK_1Q'], 'Position', pos, 'Orientation', orient);
      | 
      |         pos = get_param(    [gcb, '/fltInK_1Q'], 'Position');
      |         orient = get_param( [gcb, '/fltInK_1Q'], 'Orientation');
      |         delete_block(       [gcb, '/fltInK_1Q']);
      |         add_block('built-in/Ground', [gcb, '/fltInK_1Q'], 'Position', pos, 'Orientation', orient);
      | 
      |         pos = get_param(    [gcb, '/fltIntegPartK_1FW'], 'Position');
      |         orient = get_param( [gcb, '/fltIntegPartK_1FW'], 'Orientation');
      |         delete_block(       [gcb, '/fltIntegPartK_1FW']);
      |         add_block('built-in/Ground', [gcb, '/fltIntegPartK_1FW'], 'Position', pos, 'Orientation', orient);
      | 
      |         pos = get_param(    [gcb, '/fltInK_1FW'], 'Position');
      |         orient = get_param( [gcb, '/fltInK_1FW'], 'Orientation');
      |         delete_block(       [gcb, '/fltInK_1FW']);
      |         add_block('built-in/Ground', [gcb, '/fltInK_1FW'], 'Position', pos, 'Orientation', orient);
      | 
      |         pos = get_param(    [gcb, '/fltState'], 'Position');
      |         orient = get_param( [gcb, '/fltState'], 'Orientation');
      |         delete_block(       [gcb, '/fltState']);
      |         add_block('built-in/Ground', [gcb, '/fltState'], 'Position', pos, 'Orientation', orient);
      | 
      | 
      |         pos = get_param(    [gcb '/fltAccW_Out'], 'Position');
      |         orient = get_param( [gcb '/fltAccW_Out'], 'Orientation');
      |         delete_block(       [gcb '/fltAccW_Out']);
      |         add_block('built-in/Terminator', [gcb '/fltAccW_Out'], 'Position', pos, 'Orientation', orient);
      | 
      |         pos = get_param(    [gcb '/fltAccFW_Out'], 'Position');
      |         orient = get_param( [gcb '/fltAccFW_Out'], 'Orientation');
      |         delete_block(       [gcb '/fltAccFW_Out']);
      |         add_block('built-in/Terminator', [gcb '/fltAccFW_Out'], 'Position', pos, 'Orientation', orient);
      | 
      |         pos = get_param(    [gcb '/fltIntegPartK_1Q_Out'], 'Position');
      |         orient = get_param( [gcb '/fltIntegPartK_1Q_Out'], 'Orientation');
      |         delete_block(       [gcb '/fltIntegPartK_1Q_Out']);
      |         add_block('built-in/Terminator', [gcb '/fltIntegPartK_1Q_Out'], 'Position', pos, 'Orientation', orient);
      | 
      |         pos = get_param(    [gcb '/fltInK_1Q_Out'], 'Position');
      |         orient = get_param( [gcb '/fltInK_1Q_Out'], 'Orientation');
      |         delete_block(       [gcb '/fltInK_1Q_Out']);
      |         add_block('built-in/Terminator', [gcb '/fltInK_1Q_Out'], 'Position', pos, 'Orientation', orient);
      | 
      |         pos = get_param(    [gcb '/fltIntegPartK_1FW_Out'], 'Position');
      |         orient = get_param( [gcb '/fltIntegPartK_1FW_Out'], 'Orientation');
      |         delete_block(       [gcb '/fltIntegPartK_1FW_Out']);
      |         add_block('built-in/Terminator', [gcb '/fltIntegPartK_1FW_Out'], 'Position', pos, 'Orientation', orient);
      | 
      |         pos = get_param(    [gcb '/fltInK_1FW_Out'], 'Position');
      |         orient = get_param( [gcb '/fltInK_1FW_Out'], 'Orientation');
      |         delete_block(       [gcb '/fltInK_1FW_Out']);
      |         add_block('built-in/Terminator', [gcb '/fltInK_1FW_Out'], 'Position', pos, 'Orientation', orient);
      | 
      |         pos = get_param(    [gcb '/fltState_Out'], 'Position');
      |         orient = get_param( [gcb '/fltState_Out'], 'Orientation');
      |         delete_block(       [gcb '/fltState_Out']);
      |         add_block('built-in/Terminator', [gcb '/fltState_Out'], 'Position', pos, 'Orientation', orient);
      | 
      | 
      |         if strcmp(get_param([gcb '/fltWReqFilt'], 'BlockType'), 'Outport')
      |             pos = get_param(    [gcb '/fltWReqFilt'], 'Position');
      |             orient = get_param( [gcb '/fltWReqFilt'], 'Orientation');
      |             delete_block(       [gcb '/fltWReqFilt']);
      |             add_block('built-in/Terminator', [gcb '/fltWReqFilt'], 'Position', pos, 'Orientation', orient);
      | 
      |             pos = get_param(    [gcb '/fltWErr'], 'Position');
      |             orient = get_param( [gcb '/fltWErr'], 'Orientation');
      |             delete_block(       [gcb '/fltWErr']);
      |             add_block('built-in/Terminator', [gcb '/fltWErr'], 'Position', pos, 'Orientation', orient);
      | 
      |             pos = get_param(    [gcb '/fltIDQReqAmp'], 'Position');
      |             orient = get_param( [gcb '/fltIDQReqAmp'], 'Orientation');
      |             delete_block(       [gcb '/fltIDQReqAmp']);
      |             add_block('built-in/Terminator', [gcb '/fltIDQReqAmp'], 'Position', pos, 'Orientation', orient);
      | 
      |             pos = get_param(    [gcb '/fltWFbckFilt'], 'Position');
      |             orient = get_param( [gcb '/fltWFbckFilt'], 'Orientation');
      |             delete_block(       [gcb '/fltWFbckFilt']);
      |             add_block('built-in/Terminator', [gcb '/fltWFbckFilt'], 'Position', pos, 'Orientation', orient);
      | 
      |             pos = get_param(    [gcb '/fltIQErrSign'], 'Position');
      |             orient = get_param( [gcb '/fltIQErrSign'], 'Orientation');
      |             delete_block(       [gcb '/fltIQErrSign']);
      |             add_block('built-in/Terminator', [gcb '/fltIQErrSign'], 'Position', pos, 'Orientation', orient);
      | 
      |             pos = get_param(    [gcb '/fltFWErr'], 'Position');
      |             orient = get_param( [gcb '/fltFWErr'], 'Orientation');
      |             delete_block(       [gcb '/fltFWErr']);
      |             add_block('built-in/Terminator', [gcb '/fltFWErr'], 'Position', pos, 'Orientation', orient);
      | 
      |             pos = get_param(    [gcb '/fltIQErr'], 'Position');
      |             orient = get_param( [gcb '/fltIQErr'], 'Orientation');
      |             delete_block(       [gcb '/fltIQErr']);
      |             add_block('built-in/Terminator', [gcb '/fltIQErr'], 'Position', pos, 'Orientation', orient);
      | 
      |             pos = get_param(    [gcb '/fltUQErr'], 'Position');
      |             orient = get_param( [gcb '/fltUQErr'], 'Orientation');
      |             delete_block(       [gcb '/fltUQErr']);
      |             add_block('built-in/Terminator', [gcb '/fltUQErr'], 'Position', pos, 'Orientation', orient);
      | 
      |             pos = get_param(    [gcb '/fltFWErrFilt'], 'Position');
      |             orient = get_param( [gcb '/fltFWErrFilt'], 'Orientation');
      |             delete_block(       [gcb '/fltFWErrFilt']);
      |             add_block('built-in/Terminator', [gcb '/fltFWErrFilt'], 'Position', pos, 'Orientation', orient);
      | 
      |             pos = get_param(    [gcb '/fltFWAngle'], 'Position');
      |             orient = get_param( [gcb '/fltFWAngle'], 'Orientation');
      |             delete_block(       [gcb '/fltFWAngle']);
      |             add_block('built-in/Terminator', [gcb '/fltFWAngle'], 'Position', pos, 'Orientation', orient);
      | 
      |             pos = get_param(    [gcb '/fltFWSin'], 'Position');
      |             orient = get_param( [gcb '/fltFWSin'], 'Orientation');
      |             delete_block(       [gcb '/fltFWSin']);
      |             add_block('built-in/Terminator', [gcb '/fltFWSin'], 'Position', pos, 'Orientation', orient);
      | 
      |             pos = get_param(    [gcb '/fltFWCos'], 'Position');
      |             orient = get_param( [gcb '/fltFWCos'], 'Orientation');
      |             delete_block(       [gcb '/fltFWCos']);
      |             add_block('built-in/Terminator', [gcb '/fltFWCos'], 'Position', pos, 'Orientation', orient);
      | 
      |         end
      | 
      |         set_param([gcb '/fltVelocityReq'], 'Port', '1');
      |         set_param([gcb '/fltVelocityFbck'], 'Port', '2');
      |         set_param([gcb '/fltIQFbck'], 'Port', '3');
      |         set_param([gcb '/fltUQReq'], 'Port', '4');
      |         set_param([gcb '/fltUQLim'], 'Port', '5');
      |         set_param([gcb '/fltFilterMAWOut_preset'], 'Port', '6');
      |         set_param([gcb '/fltFilterMAFWOut_preset'], 'Port', '7');
      |         set_param([gcb '/fltControllerPIpAWQOut_preset'], 'Port', '8');
      |         set_param([gcb '/fltControllerPIpAWFWOut_preset'], 'Port', '9');
      |         set_param([gcb '/fltRampOut_preset'], 'Port', '10');
      | 
      |         set_param([gcb '/pIDQReq'], 'Port', '1');
      |         set_param([gcb '/u16LimitFlagQ'], 'Port', '2');
      |         set_param([gcb '/u16LimitFlagFW'], 'Port', '3');
      | 
      |         set_param(gcb,'MaskEnables',{'on','on','off','on','on','on','on','on','on','on','on','on','on','on','on','on'});
      | 
      |         if (posblk(4) - posblk(2)) > 275
      |           height = 275;
      |           set_param(gcb,'Position',[posblk(1), posblk(2), posblk(3), posblk(2)+height])
      |         end
      |     end
      | else
      |     % shown state variables
      |     if strcmp(get_param([gcb '/fltUmaxDivImax'], 'BlockType'), 'Ground')
      |         posblk = get_param(gcb, 'Position');
      | 
      |         pos = get_param(    [gcb, '/fltUmaxDivImax'], 'Position');
      |         orient = get_param( [gcb, '/fltUmaxDivImax'], 'Orientation');
      |         delete_block(       [gcb, '/fltUmaxDivImax']);
      |         add_block('built-in/Inport', [gcb, '/fltUmaxDivImax'], 'Position', pos, 'Orientation', orient, 'OutDataTypeStr', 'single');
      | 
      |         pos = get_param(    [gcb, '/fltLambdaW'], 'Position');
      |         orient = get_param( [gcb, '/fltLambdaW'], 'Orientation');
      |         delete_block(       [gcb, '/fltLambdaW']);
      |         add_block('built-in/Inport', [gcb, '/fltLambdaW'], 'Position', pos, 'Orientation', orient, 'OutDataTypeStr', 'single');
      | 
      |         pos = get_param(    [gcb, '/fltLambdaFW'], 'Position');
      |         orient = get_param( [gcb, '/fltLambdaFW'], 'Orientation');
      |         delete_block(       [gcb, '/fltLambdaFW']);
      |         add_block('built-in/Inport', [gcb, '/fltLambdaFW'], 'Position', pos, 'Orientation', orient, 'OutDataTypeStr', 'single');
      | 
      |         pos = get_param(    [gcb, '/fltPropGainQ'], 'Position');
      |         orient = get_param( [gcb, '/fltPropGainQ'], 'Orientation');
      |         delete_block(       [gcb, '/fltPropGainQ']);
      |         add_block('built-in/Inport', [gcb, '/fltPropGainQ'], 'Position', pos, 'Orientation', orient, 'OutDataTypeStr', 'single');
      | 
      |         pos = get_param(    [gcb, '/fltIntegGainQ'], 'Position');
      |         orient = get_param( [gcb, '/fltIntegGainQ'], 'Orientation');
      |         delete_block(       [gcb, '/fltIntegGainQ']);
      |         add_block('built-in/Inport', [gcb, '/fltIntegGainQ'], 'Position', pos, 'Orientation', orient, 'OutDataTypeStr', 'single');
      | 
      |         pos = get_param(    [gcb, '/fltLowerLimitQ'], 'Position');
      |         orient = get_param( [gcb, '/fltLowerLimitQ'], 'Orientation');
      |         delete_block(       [gcb, '/fltLowerLimitQ']);
      |         add_block('built-in/Inport', [gcb, '/fltLowerLimitQ'], 'Position', pos, 'Orientation', orient, 'OutDataTypeStr', 'single');
      | 
      |         pos = get_param(    [gcb, '/fltUpperLimitQ'], 'Position');
      |         orient = get_param( [gcb, '/fltUpperLimitQ'], 'Orientation');
      |         delete_block(       [gcb, '/fltUpperLimitQ']);
      |         add_block('built-in/Inport', [gcb, '/fltUpperLimitQ'], 'Position', pos, 'Orientation', orient, 'OutDataTypeStr', 'single');
      | 
      |         pos = get_param(    [gcb, '/fltPropGainFW'], 'Position');
      |         orient = get_param( [gcb, '/fltPropGainFW'], 'Orientation');
      |         delete_block(       [gcb, '/fltPropGainFW']);
      |         add_block('built-in/Inport', [gcb, '/fltPropGainFW'], 'Position', pos, 'Orientation', orient, 'OutDataTypeStr', 'single');
      | 
      |         pos = get_param(    [gcb, '/fltIntegGainFW'], 'Position');
      |         orient = get_param( [gcb, '/fltIntegGainFW'], 'Orientation');
      |         delete_block(       [gcb, '/fltIntegGainFW']);
      |         add_block('built-in/Inport', [gcb, '/fltIntegGainFW'], 'Position', pos, 'Orientation', orient, 'OutDataTypeStr', 'single');
      | 
      |         pos = get_param(    [gcb, '/fltLowerLimitFW'], 'Position');
      |         orient = get_param( [gcb, '/fltLowerLimitFW'], 'Orientation');
      |         delete_block(       [gcb, '/fltLowerLimitFW']);
      |         add_block('built-in/Inport', [gcb, '/fltLowerLimitFW'], 'Position', pos, 'Orientation', orient, 'OutDataTypeStr', 'single');
      | 
      |         pos = get_param(    [gcb, '/fltUpperLimitFW'], 'Position');
      |         orient = get_param( [gcb, '/fltUpperLimitFW'], 'Orientation');
      |         delete_block(       [gcb, '/fltUpperLimitFW']);
      |         add_block('built-in/Inport', [gcb, '/fltUpperLimitFW'], 'Position', pos, 'Orientation', orient, 'OutDataTypeStr', 'single');
      | 
      |         pos = get_param(    [gcb, '/fltRampUp'], 'Position');
      |         orient = get_param( [gcb, '/fltRampUp'], 'Orientation');
      |         delete_block(       [gcb, '/fltRampUp']);
      |         add_block('built-in/Inport', [gcb, '/fltRampUp'], 'Position', pos, 'Orientation', orient, 'OutDataTypeStr', 'single');
      | 
      |         pos = get_param(    [gcb, '/fltRampDown'], 'Position');
      |         orient = get_param( [gcb, '/fltRampDown'], 'Orientation');
      |         delete_block(       [gcb, '/fltRampDown']);
      |         add_block('built-in/Inport', [gcb, '/fltRampDown'], 'Position', pos, 'Orientation', orient, 'OutDataTypeStr', 'single');
      | 
      |         pos = get_param(    [gcb, '/fltIQReqK_1'], 'Position');
      |         orient = get_param( [gcb, '/fltIQReqK_1'], 'Orientation');
      |         delete_block(       [gcb, '/fltIQReqK_1']);
      |         add_block('built-in/Inport', [gcb, '/fltIQReqK_1'], 'Position', pos, 'Orientation', orient, 'OutDataTypeStr', 'single');
      | 
      |         pos = get_param(    [gcb, '/fltAccW'], 'Position');
      |         orient = get_param( [gcb, '/fltAccW'], 'Orientation');
      |         delete_block(       [gcb, '/fltAccW']);
      |         add_block('built-in/Inport', [gcb, '/fltAccW'], 'Position', pos, 'Orientation', orient, 'OutDataTypeStr', 'single');
      | 
      |         pos = get_param(    [gcb, '/fltAccFW'], 'Position');
      |         orient = get_param( [gcb, '/fltAccFW'], 'Orientation');
      |         delete_block(       [gcb, '/fltAccFW']);
      |         add_block('built-in/Inport', [gcb, '/fltAccFW'], 'Position', pos, 'Orientation', orient, 'OutDataTypeStr', 'single');
      | 
      |         pos = get_param(    [gcb, '/fltIntegPartK_1Q'], 'Position');
      |         orient = get_param( [gcb, '/fltIntegPartK_1Q'], 'Orientation');
      |         delete_block(       [gcb, '/fltIntegPartK_1Q']);
      |         add_block('built-in/Inport', [gcb, '/fltIntegPartK_1Q'], 'Position', pos, 'Orientation', orient, 'OutDataTypeStr', 'single');
      | 
      |         pos = get_param(    [gcb, '/fltInK_1Q'], 'Position');
      |         orient = get_param( [gcb, '/fltInK_1Q'], 'Orientation');
      |         delete_block(       [gcb, '/fltInK_1Q']);
      |         add_block('built-in/Inport', [gcb, '/fltInK_1Q'], 'Position', pos, 'Orientation', orient, 'OutDataTypeStr', 'single');
      | 
      |         pos = get_param(    [gcb, '/fltIntegPartK_1FW'], 'Position');
      |         orient = get_param( [gcb, '/fltIntegPartK_1FW'], 'Orientation');
      |         delete_block(       [gcb, '/fltIntegPartK_1FW']);
      |         add_block('built-in/Inport', [gcb, '/fltIntegPartK_1FW'], 'Position', pos, 'Orientation', orient, 'OutDataTypeStr', 'single');
      | 
      |         pos = get_param(    [gcb, '/fltInK_1FW'], 'Position');
      |         orient = get_param( [gcb, '/fltInK_1FW'], 'Orientation');
      |         delete_block(       [gcb, '/fltInK_1FW']);
      |         add_block('built-in/Inport', [gcb, '/fltInK_1FW'], 'Position', pos, 'Orientation', orient, 'OutDataTypeStr', 'single');
      | 
      |         pos = get_param(    [gcb, '/fltState'], 'Position');
      |         orient = get_param( [gcb, '/fltState'], 'Orientation');
      |         delete_block(       [gcb, '/fltState']);
      |         add_block('built-in/Inport', [gcb, '/fltState'], 'Position', pos, 'Orientation', orient, 'OutDataTypeStr', 'single');
      | 
      | 
      |         pos = get_param(    [gcb '/fltAccW_Out'], 'Position');
      |         orient = get_param( [gcb '/fltAccW_Out'], 'Orientation');
      |         delete_block(       [gcb '/fltAccW_Out']);
      |         add_block('built-in/Outport', [gcb '/fltAccW_Out'], 'Position', pos, 'Orientation', orient);
      | 
      |         pos = get_param(    [gcb '/fltAccFW_Out'], 'Position');
      |         orient = get_param( [gcb '/fltAccFW_Out'], 'Orientation');
      |         delete_block(       [gcb '/fltAccFW_Out']);
      |         add_block('built-in/Outport', [gcb '/fltAccFW_Out'], 'Position', pos, 'Orientation', orient);
      | 
      |         pos = get_param(    [gcb '/fltIntegPartK_1Q_Out'], 'Position');
      |         orient = get_param( [gcb '/fltIntegPartK_1Q_Out'], 'Orientation');
      |         delete_block(       [gcb '/fltIntegPartK_1Q_Out']);
      |         add_block('built-in/Outport', [gcb '/fltIntegPartK_1Q_Out'], 'Position', pos, 'Orientation', orient);
      | 
      |         pos = get_param(    [gcb '/fltInK_1Q_Out'], 'Position');
      |         orient = get_param( [gcb '/fltInK_1Q_Out'], 'Orientation');
      |         delete_block(       [gcb '/fltInK_1Q_Out']);
      |         add_block('built-in/Outport', [gcb '/fltInK_1Q_Out'], 'Position', pos, 'Orientation', orient);
      | 
      |         pos = get_param(    [gcb '/fltIntegPartK_1FW_Out'], 'Position');
      |         orient = get_param( [gcb '/fltIntegPartK_1FW_Out'], 'Orientation');
      |         delete_block(       [gcb '/fltIntegPartK_1FW_Out']);
      |         add_block('built-in/Outport', [gcb '/fltIntegPartK_1FW_Out'], 'Position', pos, 'Orientation', orient);
      | 
      |         pos = get_param(    [gcb '/fltInK_1FW_Out'], 'Position');
      |         orient = get_param( [gcb '/fltInK_1FW_Out'], 'Orientation');
      |         delete_block(       [gcb '/fltInK_1FW_Out']);
      |         add_block('built-in/Outport', [gcb '/fltInK_1FW_Out'], 'Position', pos, 'Orientation', orient);
      | 
      |         pos = get_param(    [gcb '/fltState_Out'], 'Position');
      |         orient = get_param( [gcb '/fltState_Out'], 'Orientation');
      |         delete_block(       [gcb '/fltState_Out']);
      |         add_block('built-in/Outport', [gcb '/fltState_Out'], 'Position', pos, 'Orientation', orient);
      | 
      | 
      |         if (showDebugOutputs == 2) && (strcmp(get_param([gcb '/fltWReqFilt'], 'BlockType'), 'Terminator'))
      |             pos = get_param(    [gcb '/fltWReqFilt'], 'Position');
      |             orient = get_param( [gcb '/fltWReqFilt'], 'Orientation');
      |             delete_block(       [gcb '/fltWReqFilt']);
      |             add_block('built-in/Outport', [gcb '/fltWReqFilt'], 'Position', pos, 'Orientation', orient);
      | 
      |             pos = get_param(    [gcb '/fltWErr'], 'Position');
      |             orient = get_param( [gcb '/fltWErr'], 'Orientation');
      |             delete_block(       [gcb '/fltWErr']);
      |             add_block('built-in/Outport', [gcb '/fltWErr'], 'Position', pos, 'Orientation', orient);
      | 
      |             pos = get_param(    [gcb '/fltIDQReqAmp'], 'Position');
      |             orient = get_param( [gcb '/fltIDQReqAmp'], 'Orientation');
      |             delete_block(       [gcb '/fltIDQReqAmp']);
      |             add_block('built-in/Outport', [gcb '/fltIDQReqAmp'], 'Position', pos, 'Orientation', orient);
      | 
      |             pos = get_param(    [gcb '/fltWFbckFilt'], 'Position');
      |             orient = get_param( [gcb '/fltWFbckFilt'], 'Orientation');
      |             delete_block(       [gcb '/fltWFbckFilt']);
      |             add_block('built-in/Outport', [gcb '/fltWFbckFilt'], 'Position', pos, 'Orientation', orient);
      | 
      |             pos = get_param(    [gcb '/fltIQErrSign'], 'Position');
      |             orient = get_param( [gcb '/fltIQErrSign'], 'Orientation');
      |             delete_block(       [gcb '/fltIQErrSign']);
      |             add_block('built-in/Outport', [gcb '/fltIQErrSign'], 'Position', pos, 'Orientation', orient);
      | 
      |             pos = get_param(    [gcb '/fltFWErr'], 'Position');
      |             orient = get_param( [gcb '/fltFWErr'], 'Orientation');
      |             delete_block(       [gcb '/fltFWErr']);
      |             add_block('built-in/Outport', [gcb '/fltFWErr'], 'Position', pos, 'Orientation', orient);
      | 
      |             pos = get_param(    [gcb '/fltIQErr'], 'Position');
      |             orient = get_param( [gcb '/fltIQErr'], 'Orientation');
      |             delete_block(       [gcb '/fltIQErr']);
      |             add_block('built-in/Outport', [gcb '/fltIQErr'], 'Position', pos, 'Orientation', orient);
      | 
      |             pos = get_param(    [gcb '/fltUQErr'], 'Position');
      |             orient = get_param( [gcb '/fltUQErr'], 'Orientation');
      |             delete_block(       [gcb '/fltUQErr']);
      |             add_block('built-in/Outport', [gcb '/fltUQErr'], 'Position', pos, 'Orientation', orient);
      | 
      |             pos = get_param(    [gcb '/fltFWErrFilt'], 'Position');
      |             orient = get_param( [gcb '/fltFWErrFilt'], 'Orientation');
      |             delete_block(       [gcb '/fltFWErrFilt']);
      |             add_block('built-in/Outport', [gcb '/fltFWErrFilt'], 'Position', pos, 'Orientation', orient);
      | 
      |             pos = get_param(    [gcb '/fltFWAngle'], 'Position');
      |             orient = get_param( [gcb '/fltFWAngle'], 'Orientation');
      |             delete_block(       [gcb '/fltFWAngle']);
      |             add_block('built-in/Outport', [gcb '/fltFWAngle'], 'Position', pos, 'Orientation', orient);
      | 
      |             pos = get_param(    [gcb '/fltFWSin'], 'Position');
      |             orient = get_param( [gcb '/fltFWSin'], 'Orientation');
      |             delete_block(       [gcb '/fltFWSin']);
      |             add_block('built-in/Outport', [gcb '/fltFWSin'], 'Position', pos, 'Orientation', orient);
      | 
      |             pos = get_param(    [gcb '/fltFWCos'], 'Position');
      |             orient = get_param( [gcb '/fltFWCos'], 'Orientation');
      |             delete_block(       [gcb '/fltFWCos']);
      |             add_block('built-in/Outport', [gcb '/fltFWCos'], 'Position', pos, 'Orientation', orient);
      | 
      |         end
      | 
      |         set_param([gcb '/fltVelocityReq'], 'Port', '1');
      |         set_param([gcb '/fltVelocityFbck'], 'Port', '2');
      |         set_param([gcb '/fltIQFbck'], 'Port', '3');
      |         set_param([gcb '/fltUQReq'], 'Port', '4');
      |         set_param([gcb '/fltUQLim'], 'Port', '5');
      |         set_param([gcb '/fltFilterMAWOut_preset'], 'Port', '6');
      |         set_param([gcb '/fltFilterMAFWOut_preset'], 'Port', '7');
      |         set_param([gcb '/fltControllerPIpAWQOut_preset'], 'Port', '8');
      |         set_param([gcb '/fltControllerPIpAWFWOut_preset'], 'Port', '9');
      |         set_param([gcb '/fltRampOut_preset'], 'Port', '10');
      |         set_param([gcb '/fltUmaxDivImax'], 'Port', '11');
      |         set_param([gcb '/fltLambdaW'], 'Port', '12');
      |         set_param([gcb '/fltLambdaFW'], 'Port', '13');
      |         set_param([gcb '/fltPropGainQ'], 'Port', '14');
      |         set_param([gcb '/fltIntegGainQ'], 'Port', '15');
      |         set_param([gcb '/fltLowerLimitQ'], 'Port', '16');
      |         set_param([gcb '/fltUpperLimitQ'], 'Port', '17');
      |         set_param([gcb '/fltPropGainFW'], 'Port', '18');
      |         set_param([gcb '/fltIntegGainFW'], 'Port', '19');
      |         set_param([gcb '/fltLowerLimitFW'], 'Port', '20');
      |         set_param([gcb '/fltUpperLimitFW'], 'Port', '21');
      |         set_param([gcb '/fltRampUp'], 'Port', '22');
      |         set_param([gcb '/fltRampDown'], 'Port', '23');
      |         set_param([gcb '/fltIQReqK_1'], 'Port', '24');
      |         set_param([gcb '/fltAccW'], 'Port', '25');
      |         set_param([gcb '/fltAccFW'], 'Port', '26');
      |         set_param([gcb '/fltIntegPartK_1Q'], 'Port', '27');
      |         set_param([gcb '/fltInK_1Q'], 'Port', '28');
      |         set_param([gcb '/fltIntegPartK_1FW'], 'Port', '29');
      |         set_param([gcb '/fltInK_1FW'], 'Port', '30');
      |         set_param([gcb '/fltState'], 'Port', '31');
      | 
      |         if (showDebugOutputs == 2)
      |             set_param([gcb '/pIDQReq'], 'Port', '1');
      |             set_param([gcb '/u16LimitFlagQ'], 'Port', '2');
      |             set_param([gcb '/u16LimitFlagFW'], 'Port', '3');
      |             set_param([gcb '/fltWReqFilt'], 'Port', '4');
      |             set_param([gcb '/fltWErr'], 'Port', '5');
      |             set_param([gcb '/fltIDQReqAmp'], 'Port', '6');
      |             set_param([gcb '/fltWFbckFilt'], 'Port', '7');
      |             set_param([gcb '/fltIQErrSign'], 'Port', '8');
      |             set_param([gcb '/fltFWErr'], 'Port', '9');
      |             set_param([gcb '/fltIQErr'], 'Port', '10');
      |             set_param([gcb '/fltUQErr'], 'Port', '11');
      |             set_param([gcb '/fltFWErrFilt'], 'Port', '12');
      |             set_param([gcb '/fltFWAngle'], 'Port', '13');
      |             set_param([gcb '/fltFWSin'], 'Port', '14');
      |             set_param([gcb '/fltFWCos'], 'Port', '15');
      |             set_param([gcb '/fltAccW_Out'], 'Port', '16');
      |             set_param([gcb '/fltAccFW_Out'], 'Port', '17');
      |             set_param([gcb '/fltIntegPartK_1Q_Out'], 'Port', '18');
      |             set_param([gcb '/fltInK_1Q_Out'], 'Port', '19');
      |             set_param([gcb '/fltIntegPartK_1FW_Out'], 'Port', '20');
      |             set_param([gcb '/fltInK_1FW_Out'], 'Port', '21');
      |             set_param([gcb '/fltState_Out'], 'Port', '22');
      |         else
      |             set_param([gcb '/pIDQReq'], 'Port', '1');
      |             set_param([gcb '/u16LimitFlagQ'], 'Port', '2');
      |             set_param([gcb '/u16LimitFlagFW'], 'Port', '3');
      |             set_param([gcb '/fltAccW_Out'], 'Port', '4');
      |             set_param([gcb '/fltAccFW_Out'], 'Port', '5');
      |             set_param([gcb '/fltIntegPartK_1Q_Out'], 'Port', '6');
      |             set_param([gcb '/fltInK_1Q_Out'], 'Port', '7');
      |             set_param([gcb '/fltIntegPartK_1FW_Out'], 'Port', '8');
      |             set_param([gcb '/fltInK_1FW_Out'], 'Port', '9');
      |             set_param([gcb '/fltState_Out'], 'Port', '10');
      |         end
      | 
      |         set_param(gcb,'MaskEnables',{'on','on','on','off','off','off','off','off','off','off','off','off','off','off','off','off'});
      | 
      |         if (posblk(4) - posblk(2)) < 800
      |           height = 800;
      |           set_param(gcb,'Position',[posblk(1), posblk(2), posblk(3), posblk(2)+height])
      |         end
      |     else
      |         if (showDebugOutputs == 2) && (strcmp(get_param([gcb '/fltWReqFilt'], 'BlockType'), 'Terminator'))
      |             % shown debugging outputs
      |             pos = get_param(    [gcb '/fltWReqFilt'], 'Position');
      |             orient = get_param( [gcb '/fltWReqFilt'], 'Orientation');
      |             delete_block(       [gcb '/fltWReqFilt']);
      |             add_block('built-in/Outport', [gcb '/fltWReqFilt'], 'Position', pos, 'Orientation', orient);
      | 
      |             pos = get_param(    [gcb '/fltWErr'], 'Position');
      |             orient = get_param( [gcb '/fltWErr'], 'Orientation');
      |             delete_block(       [gcb '/fltWErr']);
      |             add_block('built-in/Outport', [gcb '/fltWErr'], 'Position', pos, 'Orientation', orient);
      | 
      |             pos = get_param(    [gcb '/fltIDQReqAmp'], 'Position');
      |             orient = get_param( [gcb '/fltIDQReqAmp'], 'Orientation');
      |             delete_block(       [gcb '/fltIDQReqAmp']);
      |             add_block('built-in/Outport', [gcb '/fltIDQReqAmp'], 'Position', pos, 'Orientation', orient);
      | 
      |             pos = get_param(    [gcb '/fltWFbckFilt'], 'Position');
      |             orient = get_param( [gcb '/fltWFbckFilt'], 'Orientation');
      |             delete_block(       [gcb '/fltWFbckFilt']);
      |             add_block('built-in/Outport', [gcb '/fltWFbckFilt'], 'Position', pos, 'Orientation', orient);
      | 
      |             pos = get_param(    [gcb '/fltIQErrSign'], 'Position');
      |             orient = get_param( [gcb '/fltIQErrSign'], 'Orientation');
      |             delete_block(       [gcb '/fltIQErrSign']);
      |             add_block('built-in/Outport', [gcb '/fltIQErrSign'], 'Position', pos, 'Orientation', orient);
      | 
      |             pos = get_param(    [gcb '/fltFWErr'], 'Position');
      |             orient = get_param( [gcb '/fltFWErr'], 'Orientation');
      |             delete_block(       [gcb '/fltFWErr']);
      |             add_block('built-in/Outport', [gcb '/fltFWErr'], 'Position', pos, 'Orientation', orient);
      | 
      |             pos = get_param(    [gcb '/fltIQErr'], 'Position');
      |             orient = get_param( [gcb '/fltIQErr'], 'Orientation');
      |             delete_block(       [gcb '/fltIQErr']);
      |             add_block('built-in/Outport', [gcb '/fltIQErr'], 'Position', pos, 'Orientation', orient);
      | 
      |             pos = get_param(    [gcb '/fltUQErr'], 'Position');
      |             orient = get_param( [gcb '/fltUQErr'], 'Orientation');
      |             delete_block(       [gcb '/fltUQErr']);
      |             add_block('built-in/Outport', [gcb '/fltUQErr'], 'Position', pos, 'Orientation', orient);
      | 
      |             pos = get_param(    [gcb '/fltFWErrFilt'], 'Position');
      |             orient = get_param( [gcb '/fltFWErrFilt'], 'Orientation');
      |             delete_block(       [gcb '/fltFWErrFilt']);
      |             add_block('built-in/Outport', [gcb '/fltFWErrFilt'], 'Position', pos, 'Orientation', orient);
      | 
      |             pos = get_param(    [gcb '/fltFWAngle'], 'Position');
      |             orient = get_param( [gcb '/fltFWAngle'], 'Orientation');
      |             delete_block(       [gcb '/fltFWAngle']);
      |             add_block('built-in/Outport', [gcb '/fltFWAngle'], 'Position', pos, 'Orientation', orient);
      | 
      |             pos = get_param(    [gcb '/fltFWSin'], 'Position');
      |             orient = get_param( [gcb '/fltFWSin'], 'Orientation');
      |             delete_block(       [gcb '/fltFWSin']);
      |             add_block('built-in/Outport', [gcb '/fltFWSin'], 'Position', pos, 'Orientation', orient);
      | 
      |             pos = get_param(    [gcb '/fltFWCos'], 'Position');
      |             orient = get_param( [gcb '/fltFWCos'], 'Orientation');
      |             delete_block(       [gcb '/fltFWCos']);
      |             add_block('built-in/Outport', [gcb '/fltFWCos'], 'Position', pos, 'Orientation', orient);
      | 
      |             set_param([gcb '/pIDQReq'], 'Port', '1');
      |             set_param([gcb '/u16LimitFlagQ'], 'Port', '2');
      |             set_param([gcb '/u16LimitFlagFW'], 'Port', '3');
      |             set_param([gcb '/fltWReqFilt'], 'Port', '4');
      |             set_param([gcb '/fltWErr'], 'Port', '5');
      |             set_param([gcb '/fltIDQReqAmp'], 'Port', '6');
      |             set_param([gcb '/fltWFbckFilt'], 'Port', '7');
      |             set_param([gcb '/fltIQErrSign'], 'Port', '8');
      |             set_param([gcb '/fltFWErr'], 'Port', '9');
      |             set_param([gcb '/fltIQErr'], 'Port', '10');
      |             set_param([gcb '/fltUQErr'], 'Port', '11');
      |             set_param([gcb '/fltFWErrFilt'], 'Port', '12');
      |             set_param([gcb '/fltFWAngle'], 'Port', '13');
      |             set_param([gcb '/fltFWSin'], 'Port', '14');
      |             set_param([gcb '/fltFWCos'], 'Port', '15');
      |             set_param([gcb '/fltAccW_Out'], 'Port', '16');
      |             set_param([gcb '/fltAccFW_Out'], 'Port', '17');
      |             set_param([gcb '/fltIntegPartK_1Q_Out'], 'Port', '18');
      |             set_param([gcb '/fltInK_1Q_Out'], 'Port', '19');
      |             set_param([gcb '/fltIntegPartK_1FW_Out'], 'Port', '20');
      |             set_param([gcb '/fltInK_1FW_Out'], 'Port', '21');
      |             set_param([gcb '/fltState_Out'], 'Port', '22');
      |         elseif (showDebugOutputs == 1) && (strcmp(get_param([gcb '/fltWReqFilt'], 'BlockType'), 'Outport'))
      |             % hidden debugging outputs
      |             pos = get_param(    [gcb '/fltWReqFilt'], 'Position');
      |             orient = get_param( [gcb '/fltWReqFilt'], 'Orientation');
      |             delete_block(       [gcb '/fltWReqFilt']);
      |             add_block('built-in/Terminator', [gcb '/fltWReqFilt'], 'Position', pos, 'Orientation', orient);
      | 
      |             pos = get_param(    [gcb '/fltWErr'], 'Position');
      |             orient = get_param( [gcb '/fltWErr'], 'Orientation');
      |             delete_block(       [gcb '/fltWErr']);
      |             add_block('built-in/Terminator', [gcb '/fltWErr'], 'Position', pos, 'Orientation', orient);
      | 
      |             pos = get_param(    [gcb '/fltIDQReqAmp'], 'Position');
      |             orient = get_param( [gcb '/fltIDQReqAmp'], 'Orientation');
      |             delete_block(       [gcb '/fltIDQReqAmp']);
      |             add_block('built-in/Terminator', [gcb '/fltIDQReqAmp'], 'Position', pos, 'Orientation', orient);
      | 
      |             pos = get_param(    [gcb '/fltWFbckFilt'], 'Position');
      |             orient = get_param( [gcb '/fltWFbckFilt'], 'Orientation');
      |             delete_block(       [gcb '/fltWFbckFilt']);
      |             add_block('built-in/Terminator', [gcb '/fltWFbckFilt'], 'Position', pos, 'Orientation', orient);
      | 
      |             pos = get_param(    [gcb '/fltIQErrSign'], 'Position');
      |             orient = get_param( [gcb '/fltIQErrSign'], 'Orientation');
      |             delete_block(       [gcb '/fltIQErrSign']);
      |             add_block('built-in/Terminator', [gcb '/fltIQErrSign'], 'Position', pos, 'Orientation', orient);
      | 
      |             pos = get_param(    [gcb '/fltFWErr'], 'Position');
      |             orient = get_param( [gcb '/fltFWErr'], 'Orientation');
      |             delete_block(       [gcb '/fltFWErr']);
      |             add_block('built-in/Terminator', [gcb '/fltFWErr'], 'Position', pos, 'Orientation', orient);
      | 
      |             pos = get_param(    [gcb '/fltIQErr'], 'Position');
      |             orient = get_param( [gcb '/fltIQErr'], 'Orientation');
      |             delete_block(       [gcb '/fltIQErr']);
      |             add_block('built-in/Terminator', [gcb '/fltIQErr'], 'Position', pos, 'Orientation', orient);
      | 
      |             pos = get_param(    [gcb '/fltUQErr'], 'Position');
      |             orient = get_param( [gcb '/fltUQErr'], 'Orientation');
      |             delete_block(       [gcb '/fltUQErr']);
      |             add_block('built-in/Terminator', [gcb '/fltUQErr'], 'Position', pos, 'Orientation', orient);
      | 
      |             pos = get_param(    [gcb '/fltFWErrFilt'], 'Position');
      |             orient = get_param( [gcb '/fltFWErrFilt'], 'Orientation');
      |             delete_block(       [gcb '/fltFWErrFilt']);
      |             add_block('built-in/Terminator', [gcb '/fltFWErrFilt'], 'Position', pos, 'Orientation', orient);
      | 
      |             pos = get_param(    [gcb '/fltFWAngle'], 'Position');
      |             orient = get_param( [gcb '/fltFWAngle'], 'Orientation');
      |             delete_block(       [gcb '/fltFWAngle']);
      |             add_block('built-in/Terminator', [gcb '/fltFWAngle'], 'Position', pos, 'Orientation', orient);
      | 
      |             pos = get_param(    [gcb '/fltFWSin'], 'Position');
      |             orient = get_param( [gcb '/fltFWSin'], 'Orientation');
      |             delete_block(       [gcb '/fltFWSin']);
      |             add_block('built-in/Terminator', [gcb '/fltFWSin'], 'Position', pos, 'Orientation', orient);
      | 
      |             pos = get_param(    [gcb '/fltFWCos'], 'Position');
      |             orient = get_param( [gcb '/fltFWCos'], 'Orientation');
      |             delete_block(       [gcb '/fltFWCos']);
      |             add_block('built-in/Terminator', [gcb '/fltFWCos'], 'Position', pos, 'Orientation', orient);
      | 
      |             set_param([gcb '/pIDQReq'], 'Port', '1');
      |             set_param([gcb '/u16LimitFlagQ'], 'Port', '2');
      |             set_param([gcb '/u16LimitFlagFW'], 'Port', '3');
      |             set_param([gcb '/fltAccW_Out'], 'Port', '4');
      |             set_param([gcb '/fltAccFW_Out'], 'Port', '5');
      |             set_param([gcb '/fltIntegPartK_1Q_Out'], 'Port', '6');
      |             set_param([gcb '/fltInK_1Q_Out'], 'Port', '7');
      |             set_param([gcb '/fltIntegPartK_1FW_Out'], 'Port', '8');
      |             set_param([gcb '/fltInK_1FW_Out'], 'Port', '9');
      |             set_param([gcb '/fltState_Out'], 'Port', '10');
      |         end
      |     end
      | end
      settings: RTWSystemCode=Inline
      mask Help: web([fileparts(which('ammclib_bam_S32K14x.slx')) '/../doc/S32K14XMCLUG.pdf'], '-browser')
      mask TypeOptions showStates: Hide (faster execution) | Show (allows debugging; connect feedback loops manually)
      mask Callback showStates:
      | maskStr = get_param(gcb,'showStates');
      | if strcmp(maskStr,'Hide (faster execution)'),
      |     set_param(gcb,'MaskEnables',{'on','on','off','on','on','on','on','on','on','on','on','on','on','on','on','on'});
      | else
      |     set_param(gcb,'MaskEnables',{'on','on','on','off','off','off','off','off','off','off','off','off','off','off','off','off'});
      | end
      mask TypeOptions resetStatesEnable: Pre-set according to the first set of inputs after reset | Clear to zero
      mask TypeOptions showDebugOutputs: Hide | Show
      mask Display:
      | color('black');
      | pos = get_param(gcb, 'Position');
      | width = pos(3) - pos(1);
      | height = pos(4) - pos(2);
      | tX=width/2;
      | tY=height - 25;
      | color('black');
      | text(tX,tY, 'AMCLIB_FWSpeedLoop_FLT', 'horizontalAlignment', 'center');
      | if showStates == 2
      |   color('red');
      |   text(tX,tY - 20, ['debugging mode' char(13) char(10) '(limited performance)'], 'horizontalAlignment', 'center');
      | end
  AMCLIB_FW_FLT : Subsystem  TreatAsAtomicUnit=on  mask(AMCLIB_FW_FLT){showStates=Hide (faster execution), resetStatesEnable=Pre-set according to the first set of inputs after reset, showDebugOutputs=Hide, fltUmaxDivImax=0, fltLambda=0, fltPropGain=0, fltIntegGain=0, fltLowerLimit=0, fltUpperLimit=0}
      mask prompts: showStates "Show internal states"; resetStatesEnable "Internal state after reset"; showDebugOutputs "Show debugging outputs"; fltUmaxDivImax "fltUmaxDivImax (Maximal coil voltage divided by the maximal coil current)"; fltLambda "fltLambda (GDFLIB_FilterMA - smoothing factor)"; fltPropGain "fltPropGain (GFLIB_ControllerPIpAW - proportional gain)"; fltIntegGain "fltIntegGain (GFLIB_ControllerPIpAW - integral gain)"; fltLowerLimit "fltLowerLimit (GFLIB_ControllerPIpAW - lower limit)"; fltUpperLimit "fltUpperLimit (GFLIB_ControllerPIpAW - upper limit)"
      mask help: Field Weakening controller for the PMSM field-oriented control algorithm in single precision floating-point implementation. This block supports re-initialization of the internal state during simulation. If the block is reset, the output of the MA filter and PI controller will be aligned with the inputs fltFilterMAFWOut_preset and fltControllerPIpAWFWOut_preset. Refer to the AMMCLIB User's Guide for further details.
      mask init:
      | if ~evalin('base','exist(''tS8'',''var'')')
      |   if (2 ~= exist('SWLIBS_Typedefs.mat','file'))
      |       error('File SWLIBS_Typedefs.mat is not on the Matlab path. Please add the AMMCLIB "bam" folder in the Matlab Search Path.');
      |   else
      |       evalin('base', 'load(''SWLIBS_Typedefs.mat'')');
      |   end
      | end
      | if showStates == 1
      |     % hidden state variables
      |     if strcmp(get_param([gcb '/fltUmaxDivImax'], 'BlockType'), 'Inport')
      |         posblk = get_param(gcb, 'Position');
      | 
      |         pos = get_param(    [gcb, '/fltUmaxDivImax'], 'Position');
      |         orient = get_param( [gcb, '/fltUmaxDivImax'], 'Orientation');
      |         delete_block(       [gcb, '/fltUmaxDivImax']);
      |         add_block('built-in/Ground', [gcb, '/fltUmaxDivImax'], 'Position', pos, 'Orientation', orient);
      | 
      |         pos = get_param(    [gcb, '/fltLambda'], 'Position');
      |         orient = get_param( [gcb, '/fltLambda'], 'Orientation');
      |         delete_block(       [gcb, '/fltLambda']);
      |         add_block('built-in/Ground', [gcb, '/fltLambda'], 'Position', pos, 'Orientation', orient);
      | 
      |         pos = get_param(    [gcb, '/fltPropGain'], 'Position');
      |         orient = get_param( [gcb, '/fltPropGain'], 'Orientation');
      |         delete_block(       [gcb, '/fltPropGain']);
      |         add_block('built-in/Ground', [gcb, '/fltPropGain'], 'Position', pos, 'Orientation', orient);
      | 
      |         pos = get_param(    [gcb, '/fltIntegGain'], 'Position');
      |         orient = get_param( [gcb, '/fltIntegGain'], 'Orientation');
      |         delete_block(       [gcb, '/fltIntegGain']);
      |         add_block('built-in/Ground', [gcb, '/fltIntegGain'], 'Position', pos, 'Orientation', orient);
      | 
      |         pos = get_param(    [gcb, '/fltLowerLimit'], 'Position');
      |         orient = get_param( [gcb, '/fltLowerLimit'], 'Orientation');
      |         delete_block(       [gcb, '/fltLowerLimit']);
      |         add_block('built-in/Ground', [gcb, '/fltLowerLimit'], 'Position', pos, 'Orientation', orient);
      | 
      |         pos = get_param(    [gcb, '/fltUpperLimit'], 'Position');
      |         orient = get_param( [gcb, '/fltUpperLimit'], 'Orientation');
      |         delete_block(       [gcb, '/fltUpperLimit']);
      |         add_block('built-in/Ground', [gcb, '/fltUpperLimit'], 'Position', pos, 'Orientation', orient);
      | 
      |         pos = get_param(    [gcb, '/fltIQReqK_1'], 'Position');
      |         orient = get_param( [gcb, '/fltIQReqK_1'], 'Orientation');
      |         delete_block(       [gcb, '/fltIQReqK_1']);
      |         add_block('built-in/Ground', [gcb, '/fltIQReqK_1'], 'Position', pos, 'Orientation', orient);
      | 
      |         pos = get_param(    [gcb, '/fltAcc'], 'Position');
      |         orient = get_param( [gcb, '/fltAcc'], 'Orientation');
      |         delete_block(       [gcb, '/fltAcc']);
      |         add_block('built-in/Ground', [gcb, '/fltAcc'], 'Position', pos, 'Orientation', orient);
      | 
      |         pos = get_param(    [gcb, '/fltIntegPartK_1'], 'Position');
      |         orient = get_param( [gcb, '/fltIntegPartK_1'], 'Orientation');
      |         delete_block(       [gcb, '/fltIntegPartK_1']);
      |         add_block('built-in/Ground', [gcb, '/fltIntegPartK_1'], 'Position', pos, 'Orientation', orient);
      | 
      |         pos = get_param(    [gcb, '/fltInK_1'], 'Position');
      |         orient = get_param( [gcb, '/fltInK_1'], 'Orientation');
      |         delete_block(       [gcb, '/fltInK_1']);
      |         add_block('built-in/Ground', [gcb, '/fltInK_1'], 'Position', pos, 'Orientation', orient);
      | 
      | 
      |         pos = get_param(    [gcb '/fltAcc_Out'], 'Position');
      |         orient = get_param( [gcb '/fltAcc_Out'], 'Orientation');
      |         delete_block(       [gcb '/fltAcc_Out']);
      |         add_block('built-in/Terminator', [gcb '/fltAcc_Out'], 'Position', pos, 'Orientation', orient);
      | 
      |         pos = get_param(    [gcb '/fltIntegPartK_1_Out'], 'Position');
      |         orient = get_param( [gcb '/fltIntegPartK_1_Out'], 'Orientation');
      |         delete_block(       [gcb '/fltIntegPartK_1_Out']);
      |         add_block('built-in/Terminator', [gcb '/fltIntegPartK_1_Out'], 'Position', pos, 'Orientation', orient);
      | 
      |         pos = get_param(    [gcb '/fltInK_1_Out'], 'Position');
      |         orient = get_param( [gcb '/fltInK_1_Out'], 'Orientation');
      |         delete_block(       [gcb '/fltInK_1_Out']);
      |         add_block('built-in/Terminator', [gcb '/fltInK_1_Out'], 'Position', pos, 'Orientation', orient);
      | 
      | 
      |         if strcmp(get_param([gcb '/fltIQErrSign'], 'BlockType'), 'Outport')
      |             pos = get_param(    [gcb '/fltIQErrSign'], 'Position');
      |             orient = get_param( [gcb '/fltIQErrSign'], 'Orientation');
      |             delete_block(       [gcb '/fltIQErrSign']);
      |             add_block('built-in/Terminator', [gcb '/fltIQErrSign'], 'Position', pos, 'Orientation', orient);
      | 
      |             pos = get_param(    [gcb '/fltIQErr'], 'Position');
      |             orient = get_param( [gcb '/fltIQErr'], 'Orientation');
      |             delete_block(       [gcb '/fltIQErr']);
      |             add_block('built-in/Terminator', [gcb '/fltIQErr'], 'Position', pos, 'Orientation', orient);
      | 
      |             pos = get_param(    [gcb '/fltFWErr'], 'Position');
      |             orient = get_param( [gcb '/fltFWErr'], 'Orientation');
      |             delete_block(       [gcb '/fltFWErr']);
      |             add_block('built-in/Terminator', [gcb '/fltFWErr'], 'Position', pos, 'Orientation', orient);
      | 
      |             pos = get_param(    [gcb '/fltUQErr'], 'Position');
      |             orient = get_param( [gcb '/fltUQErr'], 'Orientation');
      |             delete_block(       [gcb '/fltUQErr']);
      |             add_block('built-in/Terminator', [gcb '/fltUQErr'], 'Position', pos, 'Orientation', orient);
      | 
      |             pos = get_param(    [gcb '/fltFWErrFilt'], 'Position');
      |             orient = get_param( [gcb '/fltFWErrFilt'], 'Orientation');
      |             delete_block(       [gcb '/fltFWErrFilt']);
      |             add_block('built-in/Terminator', [gcb '/fltFWErrFilt'], 'Position', pos, 'Orientation', orient);
      | 
      |             pos = get_param(    [gcb '/fltFWAngle'], 'Position');
      |             orient = get_param( [gcb '/fltFWAngle'], 'Orientation');
      |             delete_block(       [gcb '/fltFWAngle']);
      |             add_block('built-in/Terminator', [gcb '/fltFWAngle'], 'Position', pos, 'Orientation', orient);
      | 
      |             pos = get_param(    [gcb '/fltFWSin'], 'Position');
      |             orient = get_param( [gcb '/fltFWSin'], 'Orientation');
      |             delete_block(       [gcb '/fltFWSin']);
      |             add_block('built-in/Terminator', [gcb '/fltFWSin'], 'Position', pos, 'Orientation', orient);
      | 
      |             pos = get_param(    [gcb '/fltFWCos'], 'Position');
      |             orient = get_param( [gcb '/fltFWCos'], 'Orientation');
      |             delete_block(       [gcb '/fltFWCos']);
      |             add_block('built-in/Terminator', [gcb '/fltFWCos'], 'Position', pos, 'Orientation', orient);
      | 
      |         end
      | 
      |         set_param([gcb '/fltIDQReqAmp'], 'Port', '1');
      |         set_param([gcb '/fltVelocityFbck'], 'Port', '2');
      |         set_param([gcb '/fltIQFbck'], 'Port', '3');
      |         set_param([gcb '/fltUQReq'], 'Port', '4');
      |         set_param([gcb '/fltUQLim'], 'Port', '5');
      |         set_param([gcb '/fltFilterMAFWOut_preset'], 'Port', '6');
      |         set_param([gcb '/fltControllerPIpAWFWOut_preset'], 'Port', '7');
      | 
      |         set_param([gcb '/pIDQReq'], 'Port', '1');
      |         set_param([gcb '/u16LimitFlag'], 'Port', '2');
      | 
      |         set_param(gcb,'MaskEnables',{'on','on','off','on','on','on','on','on','on'});
      | 
      |         if (posblk(4) - posblk(2)) > 200
      |           height = 200;
      |           set_param(gcb,'Position',[posblk(1), posblk(2), posblk(3), posblk(2)+height])
      |         end
      |     end
      | else
      |     % shown state variables
      |     if strcmp(get_param([gcb '/fltUmaxDivImax'], 'BlockType'), 'Ground')
      |         posblk = get_param(gcb, 'Position');
      | 
      |         pos = get_param(    [gcb, '/fltUmaxDivImax'], 'Position');
      |         orient = get_param( [gcb, '/fltUmaxDivImax'], 'Orientation');
      |         delete_block(       [gcb, '/fltUmaxDivImax']);
      |         add_block('built-in/Inport', [gcb, '/fltUmaxDivImax'], 'Position', pos, 'Orientation', orient, 'OutDataTypeStr', 'single');
      | 
      |         pos = get_param(    [gcb, '/fltLambda'], 'Position');
      |         orient = get_param( [gcb, '/fltLambda'], 'Orientation');
      |         delete_block(       [gcb, '/fltLambda']);
      |         add_block('built-in/Inport', [gcb, '/fltLambda'], 'Position', pos, 'Orientation', orient, 'OutDataTypeStr', 'single');
      | 
      |         pos = get_param(    [gcb, '/fltPropGain'], 'Position');
      |         orient = get_param( [gcb, '/fltPropGain'], 'Orientation');
      |         delete_block(       [gcb, '/fltPropGain']);
      |         add_block('built-in/Inport', [gcb, '/fltPropGain'], 'Position', pos, 'Orientation', orient, 'OutDataTypeStr', 'single');
      | 
      |         pos = get_param(    [gcb, '/fltIntegGain'], 'Position');
      |         orient = get_param( [gcb, '/fltIntegGain'], 'Orientation');
      |         delete_block(       [gcb, '/fltIntegGain']);
      |         add_block('built-in/Inport', [gcb, '/fltIntegGain'], 'Position', pos, 'Orientation', orient, 'OutDataTypeStr', 'single');
      | 
      |         pos = get_param(    [gcb, '/fltLowerLimit'], 'Position');
      |         orient = get_param( [gcb, '/fltLowerLimit'], 'Orientation');
      |         delete_block(       [gcb, '/fltLowerLimit']);
      |         add_block('built-in/Inport', [gcb, '/fltLowerLimit'], 'Position', pos, 'Orientation', orient, 'OutDataTypeStr', 'single');
      | 
      |         pos = get_param(    [gcb, '/fltUpperLimit'], 'Position');
      |         orient = get_param( [gcb, '/fltUpperLimit'], 'Orientation');
      |         delete_block(       [gcb, '/fltUpperLimit']);
      |         add_block('built-in/Inport', [gcb, '/fltUpperLimit'], 'Position', pos, 'Orientation', orient, 'OutDataTypeStr', 'single');
      | 
      |         pos = get_param(    [gcb, '/fltIQReqK_1'], 'Position');
      |         orient = get_param( [gcb, '/fltIQReqK_1'], 'Orientation');
      |         delete_block(       [gcb, '/fltIQReqK_1']);
      |         add_block('built-in/Inport', [gcb, '/fltIQReqK_1'], 'Position', pos, 'Orientation', orient, 'OutDataTypeStr', 'single');
      | 
      |         pos = get_param(    [gcb, '/fltAcc'], 'Position');
      |         orient = get_param( [gcb, '/fltAcc'], 'Orientation');
      |         delete_block(       [gcb, '/fltAcc']);
      |         add_block('built-in/Inport', [gcb, '/fltAcc'], 'Position', pos, 'Orientation', orient, 'OutDataTypeStr', 'single');
      | 
      |         pos = get_param(    [gcb, '/fltIntegPartK_1'], 'Position');
      |         orient = get_param( [gcb, '/fltIntegPartK_1'], 'Orientation');
      |         delete_block(       [gcb, '/fltIntegPartK_1']);
      |         add_block('built-in/Inport', [gcb, '/fltIntegPartK_1'], 'Position', pos, 'Orientation', orient, 'OutDataTypeStr', 'single');
      | 
      |         pos = get_param(    [gcb, '/fltInK_1'], 'Position');
      |         orient = get_param( [gcb, '/fltInK_1'], 'Orientation');
      |         delete_block(       [gcb, '/fltInK_1']);
      |         add_block('built-in/Inport', [gcb, '/fltInK_1'], 'Position', pos, 'Orientation', orient, 'OutDataTypeStr', 'single');
      | 
      | 
      |         pos = get_param(    [gcb '/fltAcc_Out'], 'Position');
      |         orient = get_param( [gcb '/fltAcc_Out'], 'Orientation');
      |         delete_block(       [gcb '/fltAcc_Out']);
      |         add_block('built-in/Outport', [gcb '/fltAcc_Out'], 'Position', pos, 'Orientation', orient);
      | 
      |         pos = get_param(    [gcb '/fltIntegPartK_1_Out'], 'Position');
      |         orient = get_param( [gcb '/fltIntegPartK_1_Out'], 'Orientation');
      |         delete_block(       [gcb '/fltIntegPartK_1_Out']);
      |         add_block('built-in/Outport', [gcb '/fltIntegPartK_1_Out'], 'Position', pos, 'Orientation', orient);
      | 
      |         pos = get_param(    [gcb '/fltInK_1_Out'], 'Position');
      |         orient = get_param( [gcb '/fltInK_1_Out'], 'Orientation');
      |         delete_block(       [gcb '/fltInK_1_Out']);
      |         add_block('built-in/Outport', [gcb '/fltInK_1_Out'], 'Position', pos, 'Orientation', orient);
      | 
      | 
      |         if (showDebugOutputs == 2) && (strcmp(get_param([gcb '/fltIQErrSign'], 'BlockType'), 'Terminator'))
      |             pos = get_param(    [gcb '/fltIQErrSign'], 'Position');
      |             orient = get_param( [gcb '/fltIQErrSign'], 'Orientation');
      |             delete_block(       [gcb '/fltIQErrSign']);
      |             add_block('built-in/Outport', [gcb '/fltIQErrSign'], 'Position', pos, 'Orientation', orient);
      | 
      |             pos = get_param(    [gcb '/fltIQErr'], 'Position');
      |             orient = get_param( [gcb '/fltIQErr'], 'Orientation');
      |             delete_block(       [gcb '/fltIQErr']);
      |             add_block('built-in/Outport', [gcb '/fltIQErr'], 'Position', pos, 'Orientation', orient);
      | 
      |             pos = get_param(    [gcb '/fltFWErr'], 'Position');
      |             orient = get_param( [gcb '/fltFWErr'], 'Orientation');
      |             delete_block(       [gcb '/fltFWErr']);
      |             add_block('built-in/Outport', [gcb '/fltFWErr'], 'Position', pos, 'Orientation', orient);
      | 
      |             pos = get_param(    [gcb '/fltUQErr'], 'Position');
      |             orient = get_param( [gcb '/fltUQErr'], 'Orientation');
      |             delete_block(       [gcb '/fltUQErr']);
      |             add_block('built-in/Outport', [gcb '/fltUQErr'], 'Position', pos, 'Orientation', orient);
      | 
      |             pos = get_param(    [gcb '/fltFWErrFilt'], 'Position');
      |             orient = get_param( [gcb '/fltFWErrFilt'], 'Orientation');
      |             delete_block(       [gcb '/fltFWErrFilt']);
      |             add_block('built-in/Outport', [gcb '/fltFWErrFilt'], 'Position', pos, 'Orientation', orient);
      | 
      |             pos = get_param(    [gcb '/fltFWAngle'], 'Position');
      |             orient = get_param( [gcb '/fltFWAngle'], 'Orientation');
      |             delete_block(       [gcb '/fltFWAngle']);
      |             add_block('built-in/Outport', [gcb '/fltFWAngle'], 'Position', pos, 'Orientation', orient);
      | 
      |             pos = get_param(    [gcb '/fltFWSin'], 'Position');
      |             orient = get_param( [gcb '/fltFWSin'], 'Orientation');
      |             delete_block(       [gcb '/fltFWSin']);
      |             add_block('built-in/Outport', [gcb '/fltFWSin'], 'Position', pos, 'Orientation', orient);
      | 
      |             pos = get_param(    [gcb '/fltFWCos'], 'Position');
      |             orient = get_param( [gcb '/fltFWCos'], 'Orientation');
      |             delete_block(       [gcb '/fltFWCos']);
      |             add_block('built-in/Outport', [gcb '/fltFWCos'], 'Position', pos, 'Orientation', orient);
      | 
      |         end
      | 
      |         set_param([gcb '/fltIDQReqAmp'], 'Port', '1');
      |         set_param([gcb '/fltVelocityFbck'], 'Port', '2');
      |         set_param([gcb '/fltIQFbck'], 'Port', '3');
      |         set_param([gcb '/fltUQReq'], 'Port', '4');
      |         set_param([gcb '/fltUQLim'], 'Port', '5');
      |         set_param([gcb '/fltFilterMAFWOut_preset'], 'Port', '6');
      |         set_param([gcb '/fltControllerPIpAWFWOut_preset'], 'Port', '7');
      |         set_param([gcb '/fltUmaxDivImax'], 'Port', '8');
      |         set_param([gcb '/fltLambda'], 'Port', '9');
      |         set_param([gcb '/fltPropGain'], 'Port', '10');
      |         set_param([gcb '/fltIntegGain'], 'Port', '11');
      |         set_param([gcb '/fltLowerLimit'], 'Port', '12');
      |         set_param([gcb '/fltUpperLimit'], 'Port', '13');
      |         set_param([gcb '/fltIQReqK_1'], 'Port', '14');
      |         set_param([gcb '/fltAcc'], 'Port', '15');
      |         set_param([gcb '/fltIntegPartK_1'], 'Port', '16');
      |         set_param([gcb '/fltInK_1'], 'Port', '17');
      | 
      |         if (showDebugOutputs == 2)
      |             set_param([gcb '/pIDQReq'], 'Port', '1');
      |             set_param([gcb '/u16LimitFlag'], 'Port', '2');
      |             set_param([gcb '/fltIQErrSign'], 'Port', '3');
      |             set_param([gcb '/fltIQErr'], 'Port', '4');
      |             set_param([gcb '/fltFWErr'], 'Port', '5');
      |             set_param([gcb '/fltUQErr'], 'Port', '6');
      |             set_param([gcb '/fltFWErrFilt'], 'Port', '7');
      |             set_param([gcb '/fltFWAngle'], 'Port', '8');
      |             set_param([gcb '/fltFWSin'], 'Port', '9');
      |             set_param([gcb '/fltFWCos'], 'Port', '10');
      |             set_param([gcb '/fltAcc_Out'], 'Port', '11');
      |             set_param([gcb '/fltIntegPartK_1_Out'], 'Port', '12');
      |             set_param([gcb '/fltInK_1_Out'], 'Port', '13');
      |         else
      |             set_param([gcb '/pIDQReq'], 'Port', '1');
      |             set_param([gcb '/u16LimitFlag'], 'Port', '2');
      |             set_param([gcb '/fltAcc_Out'], 'Port', '3');
      |             set_param([gcb '/fltIntegPartK_1_Out'], 'Port', '4');
      |             set_param([gcb '/fltInK_1_Out'], 'Port', '5');
      |         end
      | 
      |         set_param(gcb,'MaskEnables',{'on','on','on','off','off','off','off','off','off'});
      | 
      |         if (posblk(4) - posblk(2)) < 450
      |           height = 450;
      |           set_param(gcb,'Position',[posblk(1), posblk(2), posblk(3), posblk(2)+height])
      |         end
      |     else
      |         if (showDebugOutputs == 2) && (strcmp(get_param([gcb '/fltIQErrSign'], 'BlockType'), 'Terminator'))
      |             % shown debugging outputs
      |             pos = get_param(    [gcb '/fltIQErrSign'], 'Position');
      |             orient = get_param( [gcb '/fltIQErrSign'], 'Orientation');
      |             delete_block(       [gcb '/fltIQErrSign']);
      |             add_block('built-in/Outport', [gcb '/fltIQErrSign'], 'Position', pos, 'Orientation', orient);
      | 
      |             pos = get_param(    [gcb '/fltIQErr'], 'Position');
      |             orient = get_param( [gcb '/fltIQErr'], 'Orientation');
      |             delete_block(       [gcb '/fltIQErr']);
      |             add_block('built-in/Outport', [gcb '/fltIQErr'], 'Position', pos, 'Orientation', orient);
      | 
      |             pos = get_param(    [gcb '/fltFWErr'], 'Position');
      |             orient = get_param( [gcb '/fltFWErr'], 'Orientation');
      |             delete_block(       [gcb '/fltFWErr']);
      |             add_block('built-in/Outport', [gcb '/fltFWErr'], 'Position', pos, 'Orientation', orient);
      | 
      |             pos = get_param(    [gcb '/fltUQErr'], 'Position');
      |             orient = get_param( [gcb '/fltUQErr'], 'Orientation');
      |             delete_block(       [gcb '/fltUQErr']);
      |             add_block('built-in/Outport', [gcb '/fltUQErr'], 'Position', pos, 'Orientation', orient);
      | 
      |             pos = get_param(    [gcb '/fltFWErrFilt'], 'Position');
      |             orient = get_param( [gcb '/fltFWErrFilt'], 'Orientation');
      |             delete_block(       [gcb '/fltFWErrFilt']);
      |             add_block('built-in/Outport', [gcb '/fltFWErrFilt'], 'Position', pos, 'Orientation', orient);
      | 
      |             pos = get_param(    [gcb '/fltFWAngle'], 'Position');
      |             orient = get_param( [gcb '/fltFWAngle'], 'Orientation');
      |             delete_block(       [gcb '/fltFWAngle']);
      |             add_block('built-in/Outport', [gcb '/fltFWAngle'], 'Position', pos, 'Orientation', orient);
      | 
      |             pos = get_param(    [gcb '/fltFWSin'], 'Position');
      |             orient = get_param( [gcb '/fltFWSin'], 'Orientation');
      |             delete_block(       [gcb '/fltFWSin']);
      |             add_block('built-in/Outport', [gcb '/fltFWSin'], 'Position', pos, 'Orientation', orient);
      | 
      |             pos = get_param(    [gcb '/fltFWCos'], 'Position');
      |             orient = get_param( [gcb '/fltFWCos'], 'Orientation');
      |             delete_block(       [gcb '/fltFWCos']);
      |             add_block('built-in/Outport', [gcb '/fltFWCos'], 'Position', pos, 'Orientation', orient);
      | 
      |             set_param([gcb '/pIDQReq'], 'Port', '1');
      |             set_param([gcb '/u16LimitFlag'], 'Port', '2');
      |             set_param([gcb '/fltIQErrSign'], 'Port', '3');
      |             set_param([gcb '/fltIQErr'], 'Port', '4');
      |             set_param([gcb '/fltFWErr'], 'Port', '5');
      |             set_param([gcb '/fltUQErr'], 'Port', '6');
      |             set_param([gcb '/fltFWErrFilt'], 'Port', '7');
      |             set_param([gcb '/fltFWAngle'], 'Port', '8');
      |             set_param([gcb '/fltFWSin'], 'Port', '9');
      |             set_param([gcb '/fltFWCos'], 'Port', '10');
      |             set_param([gcb '/fltAcc_Out'], 'Port', '11');
      |             set_param([gcb '/fltIntegPartK_1_Out'], 'Port', '12');
      |             set_param([gcb '/fltInK_1_Out'], 'Port', '13');
      |         elseif (showDebugOutputs == 1) && (strcmp(get_param([gcb '/fltIQErrSign'], 'BlockType'), 'Outport'))
      |             % hidden debugging outputs
      |             pos = get_param(    [gcb '/fltIQErrSign'], 'Position');
      |             orient = get_param( [gcb '/fltIQErrSign'], 'Orientation');
      |             delete_block(       [gcb '/fltIQErrSign']);
      |             add_block('built-in/Terminator', [gcb '/fltIQErrSign'], 'Position', pos, 'Orientation', orient);
      | 
      |             pos = get_param(    [gcb '/fltIQErr'], 'Position');
      |             orient = get_param( [gcb '/fltIQErr'], 'Orientation');
      |             delete_block(       [gcb '/fltIQErr']);
      |             add_block('built-in/Terminator', [gcb '/fltIQErr'], 'Position', pos, 'Orientation', orient);
      | 
      |             pos = get_param(    [gcb '/fltFWErr'], 'Position');
      |             orient = get_param( [gcb '/fltFWErr'], 'Orientation');
      |             delete_block(       [gcb '/fltFWErr']);
      |             add_block('built-in/Terminator', [gcb '/fltFWErr'], 'Position', pos, 'Orientation', orient);
      | 
      |             pos = get_param(    [gcb '/fltUQErr'], 'Position');
      |             orient = get_param( [gcb '/fltUQErr'], 'Orientation');
      |             delete_block(       [gcb '/fltUQErr']);
      |             add_block('built-in/Terminator', [gcb '/fltUQErr'], 'Position', pos, 'Orientation', orient);
      | 
      |             pos = get_param(    [gcb '/fltFWErrFilt'], 'Position');
      |             orient = get_param( [gcb '/fltFWErrFilt'], 'Orientation');
      |             delete_block(       [gcb '/fltFWErrFilt']);
      |             add_block('built-in/Terminator', [gcb '/fltFWErrFilt'], 'Position', pos, 'Orientation', orient);
      | 
      |             pos = get_param(    [gcb '/fltFWAngle'], 'Position');
      |             orient = get_param( [gcb '/fltFWAngle'], 'Orientation');
      |             delete_block(       [gcb '/fltFWAngle']);
      |             add_block('built-in/Terminator', [gcb '/fltFWAngle'], 'Position', pos, 'Orientation', orient);
      | 
      |             pos = get_param(    [gcb '/fltFWSin'], 'Position');
      |             orient = get_param( [gcb '/fltFWSin'], 'Orientation');
      |             delete_block(       [gcb '/fltFWSin']);
      |             add_block('built-in/Terminator', [gcb '/fltFWSin'], 'Position', pos, 'Orientation', orient);
      | 
      |             pos = get_param(    [gcb '/fltFWCos'], 'Position');
      |             orient = get_param( [gcb '/fltFWCos'], 'Orientation');
      |             delete_block(       [gcb '/fltFWCos']);
      |             add_block('built-in/Terminator', [gcb '/fltFWCos'], 'Position', pos, 'Orientation', orient);
      | 
      |             set_param([gcb '/pIDQReq'], 'Port', '1');
      |             set_param([gcb '/u16LimitFlag'], 'Port', '2');
      |             set_param([gcb '/fltAcc_Out'], 'Port', '3');
      |             set_param([gcb '/fltIntegPartK_1_Out'], 'Port', '4');
      |             set_param([gcb '/fltInK_1_Out'], 'Port', '5');
      |         end
      |     end
      | end
      settings: RTWSystemCode=Inline
      mask Help: web([fileparts(which('ammclib_bam_S32K14x.slx')) '/../doc/S32K14XMCLUG.pdf'], '-browser')
      mask TypeOptions showStates: Hide (faster execution) | Show (allows debugging; connect feedback loops manually)
      mask Callback showStates:
      | maskStr = get_param(gcb,'showStates');
      | if strcmp(maskStr,'Hide (faster execution)'),
      |     set_param(gcb,'MaskEnables',{'on','on','off','on','on','on','on','on','on'});
      | else
      |     set_param(gcb,'MaskEnables',{'on','on','on','off','off','off','off','off','off'});
      | end
      mask TypeOptions resetStatesEnable: Pre-set according to the first set of inputs after reset | Clear to zero
      mask TypeOptions showDebugOutputs: Hide | Show
      mask Display:
      | color('black');
      | pos = get_param(gcb, 'Position');
      | width = pos(3) - pos(1);
      | height = pos(4) - pos(2);
      | tX=width/2;
      | tY=height - 25;
      | color('black');
      | text(tX,tY, 'AMCLIB_FW_FLT', 'horizontalAlignment', 'center');
      | if showStates == 2
      |   color('red');
      |   text(tX,tY - 20, ['debugging mode' char(13) char(10) '(limited performance)'], 'horizontalAlignment', 'center');
      | end
  AMCLIB_SpeedLoop_FLT : Subsystem  TreatAsAtomicUnit=on  mask(AMCLIB_SpeedLoop_FLT){showStates=Hide (faster execution), resetStatesEnable=Pre-set according to the first set of inputs after reset, showDebugOutputs=Hide, fltLambdaW=0, fltPropGainQ=0, fltIntegGainQ=0, fltLowerLimitQ=0, fltUpperLimitQ=0, fltRampUp=0, fltRampDown=0}
      mask prompts: showStates "Show internal states"; resetStatesEnable "Internal state after reset"; showDebugOutputs "Show debugging outputs"; fltLambdaW "fltLambdaW (GDFLIB_FilterMA - smoothing factor)"; fltPropGainQ "fltPropGainQ (GFLIB_ControllerPIpAW - proportional gain)"; fltIntegGainQ "fltIntegGainQ (GFLIB_ControllerPIpAW - integral gain)"; fltLowerLimitQ "fltLowerLimitQ (GFLIB_ControllerPIpAW - lower limit)"; fltUpperLimitQ "fltUpperLimitQ (GFLIB_ControllerPIpAW - upper limit)"; fltRampUp "fltRampUp (Ramp up increment coefficient)"; fltRampDown "fltRampDown (Ramp decrement coefficient)"
      mask help: Speed loop controller for the PMSM field-oriented control algorithm in single precision floating-point implementation. This block supports re-initialization of the internal state during simulation. If the block is reset, the outputs of the MA filter, PI controller, and the ramp will be aligned with the inputs fltFilterMAWOut_preset, fltControllerPIpAWQOut_preset, and fltRampOut_preset. Refer to the AMMCLIB User's Guide for further details.
      mask init:
      | if ~evalin('base','exist(''tS8'',''var'')')
      |   if (2 ~= exist('SWLIBS_Typedefs.mat','file'))
      |       error('File SWLIBS_Typedefs.mat is not on the Matlab path. Please add the AMMCLIB "bam" folder in the Matlab Search Path.');
      |   else
      |       evalin('base', 'load(''SWLIBS_Typedefs.mat'')');
      |   end
      | end
      | if showStates == 1
      |     % hidden state variables
      |     if strcmp(get_param([gcb '/fltLambdaW'], 'BlockType'), 'Inport')
      |         posblk = get_param(gcb, 'Position');
      | 
      |         pos = get_param(    [gcb, '/fltLambdaW'], 'Position');
      |         orient = get_param( [gcb, '/fltLambdaW'], 'Orientation');
      |         delete_block(       [gcb, '/fltLambdaW']);
      |         add_block('built-in/Ground', [gcb, '/fltLambdaW'], 'Position', pos, 'Orientation', orient);
      | 
      |         pos = get_param(    [gcb, '/fltPropGainQ'], 'Position');
      |         orient = get_param( [gcb, '/fltPropGainQ'], 'Orientation');
      |         delete_block(       [gcb, '/fltPropGainQ']);
      |         add_block('built-in/Ground', [gcb, '/fltPropGainQ'], 'Position', pos, 'Orientation', orient);
      | 
      |         pos = get_param(    [gcb, '/fltIntegGainQ'], 'Position');
      |         orient = get_param( [gcb, '/fltIntegGainQ'], 'Orientation');
      |         delete_block(       [gcb, '/fltIntegGainQ']);
      |         add_block('built-in/Ground', [gcb, '/fltIntegGainQ'], 'Position', pos, 'Orientation', orient);
      | 
      |         pos = get_param(    [gcb, '/fltLowerLimitQ'], 'Position');
      |         orient = get_param( [gcb, '/fltLowerLimitQ'], 'Orientation');
      |         delete_block(       [gcb, '/fltLowerLimitQ']);
      |         add_block('built-in/Ground', [gcb, '/fltLowerLimitQ'], 'Position', pos, 'Orientation', orient);
      | 
      |         pos = get_param(    [gcb, '/fltUpperLimitQ'], 'Position');
      |         orient = get_param( [gcb, '/fltUpperLimitQ'], 'Orientation');
      |         delete_block(       [gcb, '/fltUpperLimitQ']);
      |         add_block('built-in/Ground', [gcb, '/fltUpperLimitQ'], 'Position', pos, 'Orientation', orient);
      | 
      |         pos = get_param(    [gcb, '/fltRampUp'], 'Position');
      |         orient = get_param( [gcb, '/fltRampUp'], 'Orientation');
      |         delete_block(       [gcb, '/fltRampUp']);
      |         add_block('built-in/Ground', [gcb, '/fltRampUp'], 'Position', pos, 'Orientation', orient);
      | 
      |         pos = get_param(    [gcb, '/fltRampDown'], 'Position');
      |         orient = get_param( [gcb, '/fltRampDown'], 'Orientation');
      |         delete_block(       [gcb, '/fltRampDown']);
      |         add_block('built-in/Ground', [gcb, '/fltRampDown'], 'Position', pos, 'Orientation', orient);
      | 
      |         pos = get_param(    [gcb, '/fltAccW'], 'Position');
      |         orient = get_param( [gcb, '/fltAccW'], 'Orientation');
      |         delete_block(       [gcb, '/fltAccW']);
      |         add_block('built-in/Ground', [gcb, '/fltAccW'], 'Position', pos, 'Orientation', orient);
      | 
      |         pos = get_param(    [gcb, '/fltIntegPartK_1Q'], 'Position');
      |         orient = get_param( [gcb, '/fltIntegPartK_1Q'], 'Orientation');
      |         delete_block(       [gcb, '/fltIntegPartK_1Q']);
      |         add_block('built-in/Ground', [gcb, '/fltIntegPartK_1Q'], 'Position', pos, 'Orientation', orient);
      | 
      |         pos = get_param(    [gcb, '/fltInK_1Q'], 'Position');
      |         orient = get_param( [gcb, '/fltInK_1Q'], 'Orientation');
      |         delete_block(       [gcb, '/fltInK_1Q']);
      |         add_block('built-in/Ground', [gcb, '/fltInK_1Q'], 'Position', pos, 'Orientation', orient);
      | 
      |         pos = get_param(    [gcb, '/fltState'], 'Position');
      |         orient = get_param( [gcb, '/fltState'], 'Orientation');
      |         delete_block(       [gcb, '/fltState']);
      |         add_block('built-in/Ground', [gcb, '/fltState'], 'Position', pos, 'Orientation', orient);
      | 
      | 
      |         pos = get_param(    [gcb '/fltAccW_Out'], 'Position');
      |         orient = get_param( [gcb '/fltAccW_Out'], 'Orientation');
      |         delete_block(       [gcb '/fltAccW_Out']);
      |         add_block('built-in/Terminator', [gcb '/fltAccW_Out'], 'Position', pos, 'Orientation', orient);
      | 
      |         pos = get_param(    [gcb '/fltIntegPartK_1Q_Out'], 'Position');
      |         orient = get_param( [gcb '/fltIntegPartK_1Q_Out'], 'Orientation');
      |         delete_block(       [gcb '/fltIntegPartK_1Q_Out']);
      |         add_block('built-in/Terminator', [gcb '/fltIntegPartK_1Q_Out'], 'Position', pos, 'Orientation', orient);
      | 
      |         pos = get_param(    [gcb '/fltInK_1Q_Out'], 'Position');
      |         orient = get_param( [gcb '/fltInK_1Q_Out'], 'Orientation');
      |         delete_block(       [gcb '/fltInK_1Q_Out']);
      |         add_block('built-in/Terminator', [gcb '/fltInK_1Q_Out'], 'Position', pos, 'Orientation', orient);
      | 
      |         pos = get_param(    [gcb '/fltState_Out'], 'Position');
      |         orient = get_param( [gcb '/fltState_Out'], 'Orientation');
      |         delete_block(       [gcb '/fltState_Out']);
      |         add_block('built-in/Terminator', [gcb '/fltState_Out'], 'Position', pos, 'Orientation', orient);
      | 
      | 
      |         if strcmp(get_param([gcb '/fltWReqFilt'], 'BlockType'), 'Outport')
      |             pos = get_param(    [gcb '/fltWReqFilt'], 'Position');
      |             orient = get_param( [gcb '/fltWReqFilt'], 'Orientation');
      |             delete_block(       [gcb '/fltWReqFilt']);
      |             add_block('built-in/Terminator', [gcb '/fltWReqFilt'], 'Position', pos, 'Orientation', orient);
      | 
      |             pos = get_param(    [gcb '/fltWErr'], 'Position');
      |             orient = get_param( [gcb '/fltWErr'], 'Orientation');
      |             delete_block(       [gcb '/fltWErr']);
      |             add_block('built-in/Terminator', [gcb '/fltWErr'], 'Position', pos, 'Orientation', orient);
      | 
      |             pos = get_param(    [gcb '/fltWFbckFilt'], 'Position');
      |             orient = get_param( [gcb '/fltWFbckFilt'], 'Orientation');
      |             delete_block(       [gcb '/fltWFbckFilt']);
      |             add_block('built-in/Terminator', [gcb '/fltWFbckFilt'], 'Position', pos, 'Orientation', orient);
      | 
      |         end
      | 
      |         set_param([gcb '/fltVelocityReq'], 'Port', '1');
      |         set_param([gcb '/fltVelocityFbck'], 'Port', '2');
      |         set_param([gcb '/fltFilterMAWOut_preset'], 'Port', '3');
      |         set_param([gcb '/fltControllerPIpAWQOut_preset'], 'Port', '4');
      |         set_param([gcb '/fltRampOut_preset'], 'Port', '5');
      | 
      |         set_param([gcb '/pIDQReq'], 'Port', '1');
      |         set_param([gcb '/u16LimitFlagQ'], 'Port', '2');
      | 
      |         set_param(gcb,'MaskEnables',{'on','on','off','on','on','on','on','on','on','on'});
      | 
      |         if (posblk(4) - posblk(2)) > 150
      |           height = 150;
      |           set_param(gcb,'Position',[posblk(1), posblk(2), posblk(3), posblk(2)+height])
      |         end
      |     end
      | else
      |     % shown state variables
      |     if strcmp(get_param([gcb '/fltLambdaW'], 'BlockType'), 'Ground')
      |         posblk = get_param(gcb, 'Position');
      | 
      |         pos = get_param(    [gcb, '/fltLambdaW'], 'Position');
      |         orient = get_param( [gcb, '/fltLambdaW'], 'Orientation');
      |         delete_block(       [gcb, '/fltLambdaW']);
      |         add_block('built-in/Inport', [gcb, '/fltLambdaW'], 'Position', pos, 'Orientation', orient, 'OutDataTypeStr', 'single');
      | 
      |         pos = get_param(    [gcb, '/fltPropGainQ'], 'Position');
      |         orient = get_param( [gcb, '/fltPropGainQ'], 'Orientation');
      |         delete_block(       [gcb, '/fltPropGainQ']);
      |         add_block('built-in/Inport', [gcb, '/fltPropGainQ'], 'Position', pos, 'Orientation', orient, 'OutDataTypeStr', 'single');
      | 
      |         pos = get_param(    [gcb, '/fltIntegGainQ'], 'Position');
      |         orient = get_param( [gcb, '/fltIntegGainQ'], 'Orientation');
      |         delete_block(       [gcb, '/fltIntegGainQ']);
      |         add_block('built-in/Inport', [gcb, '/fltIntegGainQ'], 'Position', pos, 'Orientation', orient, 'OutDataTypeStr', 'single');
      | 
      |         pos = get_param(    [gcb, '/fltLowerLimitQ'], 'Position');
      |         orient = get_param( [gcb, '/fltLowerLimitQ'], 'Orientation');
      |         delete_block(       [gcb, '/fltLowerLimitQ']);
      |         add_block('built-in/Inport', [gcb, '/fltLowerLimitQ'], 'Position', pos, 'Orientation', orient, 'OutDataTypeStr', 'single');
      | 
      |         pos = get_param(    [gcb, '/fltUpperLimitQ'], 'Position');
      |         orient = get_param( [gcb, '/fltUpperLimitQ'], 'Orientation');
      |         delete_block(       [gcb, '/fltUpperLimitQ']);
      |         add_block('built-in/Inport', [gcb, '/fltUpperLimitQ'], 'Position', pos, 'Orientation', orient, 'OutDataTypeStr', 'single');
      | 
      |         pos = get_param(    [gcb, '/fltRampUp'], 'Position');
      |         orient = get_param( [gcb, '/fltRampUp'], 'Orientation');
      |         delete_block(       [gcb, '/fltRampUp']);
      |         add_block('built-in/Inport', [gcb, '/fltRampUp'], 'Position', pos, 'Orientation', orient, 'OutDataTypeStr', 'single');
      | 
      |         pos = get_param(    [gcb, '/fltRampDown'], 'Position');
      |         orient = get_param( [gcb, '/fltRampDown'], 'Orientation');
      |         delete_block(       [gcb, '/fltRampDown']);
      |         add_block('built-in/Inport', [gcb, '/fltRampDown'], 'Position', pos, 'Orientation', orient, 'OutDataTypeStr', 'single');
      | 
      |         pos = get_param(    [gcb, '/fltAccW'], 'Position');
      |         orient = get_param( [gcb, '/fltAccW'], 'Orientation');
      |         delete_block(       [gcb, '/fltAccW']);
      |         add_block('built-in/Inport', [gcb, '/fltAccW'], 'Position', pos, 'Orientation', orient, 'OutDataTypeStr', 'single');
      | 
      |         pos = get_param(    [gcb, '/fltIntegPartK_1Q'], 'Position');
      |         orient = get_param( [gcb, '/fltIntegPartK_1Q'], 'Orientation');
      |         delete_block(       [gcb, '/fltIntegPartK_1Q']);
      |         add_block('built-in/Inport', [gcb, '/fltIntegPartK_1Q'], 'Position', pos, 'Orientation', orient, 'OutDataTypeStr', 'single');
      | 
      |         pos = get_param(    [gcb, '/fltInK_1Q'], 'Position');
      |         orient = get_param( [gcb, '/fltInK_1Q'], 'Orientation');
      |         delete_block(       [gcb, '/fltInK_1Q']);
      |         add_block('built-in/Inport', [gcb, '/fltInK_1Q'], 'Position', pos, 'Orientation', orient, 'OutDataTypeStr', 'single');
      | 
      |         pos = get_param(    [gcb, '/fltState'], 'Position');
      |         orient = get_param( [gcb, '/fltState'], 'Orientation');
      |         delete_block(       [gcb, '/fltState']);
      |         add_block('built-in/Inport', [gcb, '/fltState'], 'Position', pos, 'Orientation', orient, 'OutDataTypeStr', 'single');
      | 
      | 
      |         pos = get_param(    [gcb '/fltAccW_Out'], 'Position');
      |         orient = get_param( [gcb '/fltAccW_Out'], 'Orientation');
      |         delete_block(       [gcb '/fltAccW_Out']);
      |         add_block('built-in/Outport', [gcb '/fltAccW_Out'], 'Position', pos, 'Orientation', orient);
      | 
      |         pos = get_param(    [gcb '/fltIntegPartK_1Q_Out'], 'Position');
      |         orient = get_param( [gcb '/fltIntegPartK_1Q_Out'], 'Orientation');
      |         delete_block(       [gcb '/fltIntegPartK_1Q_Out']);
      |         add_block('built-in/Outport', [gcb '/fltIntegPartK_1Q_Out'], 'Position', pos, 'Orientation', orient);
      | 
      |         pos = get_param(    [gcb '/fltInK_1Q_Out'], 'Position');
      |         orient = get_param( [gcb '/fltInK_1Q_Out'], 'Orientation');
      |         delete_block(       [gcb '/fltInK_1Q_Out']);
      |         add_block('built-in/Outport', [gcb '/fltInK_1Q_Out'], 'Position', pos, 'Orientation', orient);
      | 
      |         pos = get_param(    [gcb '/fltState_Out'], 'Position');
      |         orient = get_param( [gcb '/fltState_Out'], 'Orientation');
      |         delete_block(       [gcb '/fltState_Out']);
      |         add_block('built-in/Outport', [gcb '/fltState_Out'], 'Position', pos, 'Orientation', orient);
      | 
      | 
      |         if (showDebugOutputs == 2) && (strcmp(get_param([gcb '/fltWReqFilt'], 'BlockType'), 'Terminator'))
      |             pos = get_param(    [gcb '/fltWReqFilt'], 'Position');
      |             orient = get_param( [gcb '/fltWReqFilt'], 'Orientation');
      |             delete_block(       [gcb '/fltWReqFilt']);
      |             add_block('built-in/Outport', [gcb '/fltWReqFilt'], 'Position', pos, 'Orientation', orient);
      | 
      |             pos = get_param(    [gcb '/fltWErr'], 'Position');
      |             orient = get_param( [gcb '/fltWErr'], 'Orientation');
      |             delete_block(       [gcb '/fltWErr']);
      |             add_block('built-in/Outport', [gcb '/fltWErr'], 'Position', pos, 'Orientation', orient);
      | 
      |             pos = get_param(    [gcb '/fltWFbckFilt'], 'Position');
      |             orient = get_param( [gcb '/fltWFbckFilt'], 'Orientation');
      |             delete_block(       [gcb '/fltWFbckFilt']);
      |             add_block('built-in/Outport', [gcb '/fltWFbckFilt'], 'Position', pos, 'Orientation', orient);
      | 
      |         end
      | 
      |         set_param([gcb '/fltVelocityReq'], 'Port', '1');
      |         set_param([gcb '/fltVelocityFbck'], 'Port', '2');
      |         set_param([gcb '/fltFilterMAWOut_preset'], 'Port', '3');
      |         set_param([gcb '/fltControllerPIpAWQOut_preset'], 'Port', '4');
      |         set_param([gcb '/fltRampOut_preset'], 'Port', '5');
      |         set_param([gcb '/fltLambdaW'], 'Port', '6');
      |         set_param([gcb '/fltPropGainQ'], 'Port', '7');
      |         set_param([gcb '/fltIntegGainQ'], 'Port', '8');
      |         set_param([gcb '/fltLowerLimitQ'], 'Port', '9');
      |         set_param([gcb '/fltUpperLimitQ'], 'Port', '10');
      |         set_param([gcb '/fltRampUp'], 'Port', '11');
      |         set_param([gcb '/fltRampDown'], 'Port', '12');
      |         set_param([gcb '/fltAccW'], 'Port', '13');
      |         set_param([gcb '/fltIntegPartK_1Q'], 'Port', '14');
      |         set_param([gcb '/fltInK_1Q'], 'Port', '15');
      |         set_param([gcb '/fltState'], 'Port', '16');
      | 
      |         if (showDebugOutputs == 2)
      |             set_param([gcb '/pIDQReq'], 'Port', '1');
      |             set_param([gcb '/u16LimitFlagQ'], 'Port', '2');
      |             set_param([gcb '/fltWReqFilt'], 'Port', '3');
      |             set_param([gcb '/fltWErr'], 'Port', '4');
      |             set_param([gcb '/fltWFbckFilt'], 'Port', '5');
      |             set_param([gcb '/fltAccW_Out'], 'Port', '6');
      |             set_param([gcb '/fltIntegPartK_1Q_Out'], 'Port', '7');
      |             set_param([gcb '/fltInK_1Q_Out'], 'Port', '8');
      |             set_param([gcb '/fltState_Out'], 'Port', '9');
      |         else
      |             set_param([gcb '/pIDQReq'], 'Port', '1');
      |             set_param([gcb '/u16LimitFlagQ'], 'Port', '2');
      |             set_param([gcb '/fltAccW_Out'], 'Port', '3');
      |             set_param([gcb '/fltIntegPartK_1Q_Out'], 'Port', '4');
      |             set_param([gcb '/fltInK_1Q_Out'], 'Port', '5');
      |             set_param([gcb '/fltState_Out'], 'Port', '6');
      |         end
      | 
      |         set_param(gcb,'MaskEnables',{'on','on','on','off','off','off','off','off','off','off'});
      | 
      |         if (posblk(4) - posblk(2)) < 425
      |           height = 425;
      |           set_param(gcb,'Position',[posblk(1), posblk(2), posblk(3), posblk(2)+height])
      |         end
      |     else
      |         if (showDebugOutputs == 2) && (strcmp(get_param([gcb '/fltWReqFilt'], 'BlockType'), 'Terminator'))
      |             % shown debugging outputs
      |             pos = get_param(    [gcb '/fltWReqFilt'], 'Position');
      |             orient = get_param( [gcb '/fltWReqFilt'], 'Orientation');
      |             delete_block(       [gcb '/fltWReqFilt']);
      |             add_block('built-in/Outport', [gcb '/fltWReqFilt'], 'Position', pos, 'Orientation', orient);
      | 
      |             pos = get_param(    [gcb '/fltWErr'], 'Position');
      |             orient = get_param( [gcb '/fltWErr'], 'Orientation');
      |             delete_block(       [gcb '/fltWErr']);
      |             add_block('built-in/Outport', [gcb '/fltWErr'], 'Position', pos, 'Orientation', orient);
      | 
      |             pos = get_param(    [gcb '/fltWFbckFilt'], 'Position');
      |             orient = get_param( [gcb '/fltWFbckFilt'], 'Orientation');
      |             delete_block(       [gcb '/fltWFbckFilt']);
      |             add_block('built-in/Outport', [gcb '/fltWFbckFilt'], 'Position', pos, 'Orientation', orient);
      | 
      |             set_param([gcb '/pIDQReq'], 'Port', '1');
      |             set_param([gcb '/u16LimitFlagQ'], 'Port', '2');
      |             set_param([gcb '/fltWReqFilt'], 'Port', '3');
      |             set_param([gcb '/fltWErr'], 'Port', '4');
      |             set_param([gcb '/fltWFbckFilt'], 'Port', '5');
      |             set_param([gcb '/fltAccW_Out'], 'Port', '6');
      |             set_param([gcb '/fltIntegPartK_1Q_Out'], 'Port', '7');
      |             set_param([gcb '/fltInK_1Q_Out'], 'Port', '8');
      |             set_param([gcb '/fltState_Out'], 'Port', '9');
      |         elseif (showDebugOutputs == 1) && (strcmp(get_param([gcb '/fltWReqFilt'], 'BlockType'), 'Outport'))
      |             % hidden debugging outputs
      |             pos = get_param(    [gcb '/fltWReqFilt'], 'Position');
      |             orient = get_param( [gcb '/fltWReqFilt'], 'Orientation');
      |             delete_block(       [gcb '/fltWReqFilt']);
      |             add_block('built-in/Terminator', [gcb '/fltWReqFilt'], 'Position', pos, 'Orientation', orient);
      | 
      |             pos = get_param(    [gcb '/fltWErr'], 'Position');
      |             orient = get_param( [gcb '/fltWErr'], 'Orientation');
      |             delete_block(       [gcb '/fltWErr']);
      |             add_block('built-in/Terminator', [gcb '/fltWErr'], 'Position', pos, 'Orientation', orient);
      | 
      |             pos = get_param(    [gcb '/fltWFbckFilt'], 'Position');
      |             orient = get_param( [gcb '/fltWFbckFilt'], 'Orientation');
      |             delete_block(       [gcb '/fltWFbckFilt']);
      |             add_block('built-in/Terminator', [gcb '/fltWFbckFilt'], 'Position', pos, 'Orientation', orient);
      | 
      |             set_param([gcb '/pIDQReq'], 'Port', '1');
      |             set_param([gcb '/u16LimitFlagQ'], 'Port', '2');
      |             set_param([gcb '/fltAccW_Out'], 'Port', '3');
      |             set_param([gcb '/fltIntegPartK_1Q_Out'], 'Port', '4');
      |             set_param([gcb '/fltInK_1Q_Out'], 'Port', '5');
      |             set_param([gcb '/fltState_Out'], 'Port', '6');
      |         end
      |     end
      | end
      settings: RTWSystemCode=Inline
      mask Help: web([fileparts(which('ammclib_bam_S32K14x.slx')) '/../doc/S32K14XMCLUG.pdf'], '-browser')
      mask TypeOptions showStates: Hide (faster execution) | Show (allows debugging; connect feedback loops manually)
      mask Callback showStates:
      | maskStr = get_param(gcb,'showStates');
      | if strcmp(maskStr,'Hide (faster execution)'),
      |     set_param(gcb,'MaskEnables',{'on','on','off','on','on','on','on','on','on','on'});
      | else
      |     set_param(gcb,'MaskEnables',{'on','on','on','off','off','off','off','off','off','off'});
      | end
